simulink library "inp"  (R2021b)
settings: Solver=VariableStepAuto  StartTime=0.0  StopTime=10.0  RelTol=1e-3
undefined symbols (not defined in the file): C_TASK_5MS_S, FALSE, KINP_AcoreReadyToSlp_flg_ovrdflg, KINP_AcoreReadyToSlp_flg_ovrdval, KINP_AllowMovThd_OTA_enum_ovrdflg, KINP_AllowMovThd_OTA_enum_ovrdval, KINP_APSAngleTarget_Deg_ovrdflg, KINP_APSAngleTarget_Deg_ovrdval, KINP_APSDecReq_mps2_ovrdflg, KINP_APSDecReq_mps2_ovrdval, KINP_APSDecReqA_flg_ovrdflg, KINP_APSDecReqA_flg_ovrdval, KINP_APSDFLL_cm_ovrdflg, KINP_APSDFLL_cm_ovrdval, KINP_APSDFLR_cm_ovrdflg, KINP_APSDFLR_cm_ovrdval, KINP_APSDRLL_cm_ovrdflg, KINP_APSDRLL_cm_ovrdval, KINP_APSDRLR_cm_ovrdflg, KINP_APSDRLR_cm_ovrdval, KINP_APSExitCondition_enum_ovrdflg, KINP_APSExitCondition_enum_ovrdval, KINP_APSHWVer_enum_ovrdflg, KINP_APSHWVer_enum_ovrdval, KINP_APSProgressPCT_pct_ovrdflg, KINP_APSProgressPCT_pct_ovrdval, KINP_APSReq_enum_ovrdflg, KINP_APSReq_enum_ovrdval, KINP_APSRQDisplay_enum_ovrdflg, KINP_APSRQDisplay_enum_ovrdval, KINP_APSRqEPASCtrl_flg_ovrdflg, KINP_APSRqEPASCtrl_flg_ovrdval, KINP_APSShiftPosnReq_enum_ovrdval, KINP_APSShiftPosnReq_enum_ovrflg, KINP_APSSpeedCMD_kph_ovrdval, KINP_APSSpeedCMD_kph_ovrflg, KINP_APSStaSystem_enum_ovrdflg, KINP_APSStaSystem_enum_ovrdval, KINP_APSSWVer_enum_ovrdflg, KINP_APSSWVer_enum_ovrdval, KINP_APSVMCReqA_flg_ovrdval, KINP_APSVMCReqA_flg_ovrflg, KINP_APSVRqEPASCtrl_flg_ovrdflg, KINP_APSVRqEPASCtrl_flg_ovrdval, KINP_AuxBattVolmV_mV_ovrdflg, KINP_AuxBattVolmV_mV_ovrdval, KINP_CAASSta_enum_ovrdflg, KINP_CAASSta_enum_ovrdval, KINP_CAASVMCReqA_flg_ovrdval, KINP_CAASVMCReqA_flg_ovrflg, KINP_Chime_enum_ovrdflg, KINP_Chime_enum_ovrdval, KINP_ClearDTCcmd_flg_ovrdflg, KINP_ClearDTCcmd_flg_ovrdval, KINP_EvccAplusPwrUpReq_flg_ovrdflg, KINP_EvccAplusPwrUpReq_flg_ovrdval, KINP_LFID_raw_ovrdval, KINP_LFID_raw_ovrflg, KINP_LRID_raw_ovrdval, KINP_MemOffsetAccX_raw16_ovrdflg ... (+118)
libraries: FVT_lib x503, hcu_lib x1
(part 9 of 16)

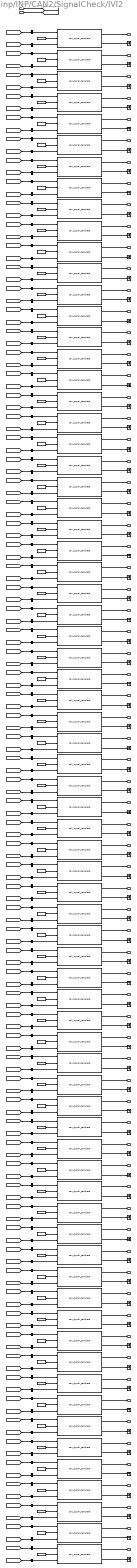
== system inp/INP/CAN2/SignalCheck/IVI2 ==
  BHAL_outputs : Inport
  inp_CanValid_bus : Inport  Port=2
  ACChgCurSet : FVT_lib/inp/can_signal_template  SystemSampleTime=-1  VariantActivationTime=update diagram  Latency=0  AutoFrameSizeCalculation=off
      link override defval: Value=KINP_ACChgCurSet_A_defval
      link override ovrdflg: Value=KINP_ACChgCurSet_A_ovrdflg
      link override ovrdval: Value=KINP_ACChgCurSet_A_ovrdval
  AVMErrSTA : FVT_lib/inp/can_signal_template  SystemSampleTime=-1  VariantActivationTime=update diagram  Latency=0  AutoFrameSizeCalculation=off
      link override defval: Value=KINP_AVMErrSTA_flg_defval
      link override ovrdflg: Value=KINP_AVMErrSTA_flg_ovrdflg
      link override ovrdval: Value=KINP_AVMErrSTA_flg_ovrdval
  AVMOFFRecButt : FVT_lib/inp/can_signal_template  SystemSampleTime=-1  VariantActivationTime=update diagram  Latency=0  AutoFrameSizeCalculation=off
      link override defval: Value=KINP_AVMOFFRecButt_flg_defval
      link override ovrdflg: Value=KINP_AVMOFFRecButt_flg_ovrdflg
      link override ovrdval: Value=KINP_AVMOFFRecButt_flg_ovrdval
  AVMParkingmode : FVT_lib/inp/can_signal_template  SystemSampleTime=-1  VariantActivationTime=update diagram  Latency=0  AutoFrameSizeCalculation=off
      link override defval: Value=KINP_AVMParkingmode_enum_defval
      link override ovrdflg: Value=KINP_AVMParkingmode_enum_ovrdflg
      link override ovrdval: Value=KINP_AVMParkingmode_enum_ovrdval
  AVMparkingcancel : FVT_lib/inp/can_signal_template  SystemSampleTime=-1  VariantActivationTime=update diagram  Latency=0  AutoFrameSizeCalculation=off
      link override defval: Value=KINP_AVMparkingcancel_enum_defval
      link override ovrdflg: Value=KINP_AVMparkingcancel_enum_ovrdflg
      link override ovrdval: Value=KINP_AVMparkingcancel_enum_ovrdval
  AVMparkingexcute : FVT_lib/inp/can_signal_template  SystemSampleTime=-1  VariantActivationTime=update diagram  Latency=0  AutoFrameSizeCalculation=off
      link override defval: Value=KINP_AVMparkingexcute_enum_defval
      link override ovrdflg: Value=KINP_AVMparkingexcute_enum_ovrdflg
      link override ovrdval: Value=KINP_AVMparkingexcute_enum_ovrdval
  CAASSw : FVT_lib/inp/can_signal_template  SystemSampleTime=-1  VariantActivationTime=update diagram  Latency=0  AutoFrameSizeCalculation=off
      link override defval: Value=KINP_CAASSw_enum_defval
      link override ovrdflg: Value=KINP_CAASSw_enum_ovrdflg
      link override ovrdval: Value=KINP_CAASSw_enum_ovrdval
  CDLLockButt : FVT_lib/inp/can_signal_template  SystemSampleTime=-1  VariantActivationTime=update diagram  Latency=0  AutoFrameSizeCalculation=off
      link override defval: Value=KINP_CDLLockButt_flg_defval
      link override ovrdflg: Value=KINP_CDLLockButt_flg_ovrdflg
      link override ovrdval: Value=KINP_CDLLockButt_flg_ovrdval
  CDLUnlockButt : FVT_lib/inp/can_signal_template  SystemSampleTime=-1  VariantActivationTime=update diagram  Latency=0  AutoFrameSizeCalculation=off
      link override defval: Value=KINP_CDLUnlockButt_flg_defval
      link override ovrdflg: Value=KINP_CDLUnlockButt_flg_ovrdflg
      link override ovrdval: Value=KINP_CDLUnlockButt_flg_ovrdval
  DSEATantiset : FVT_lib/inp/can_signal_template  SystemSampleTime=-1  VariantActivationTime=update diagram  Latency=0  AutoFrameSizeCalculation=off
      link override defval: Value=KINP_DSEATantiset_flg_defval
      link override ovrdflg: Value=KINP_DSEATantiset_flg_ovrdflg
      link override ovrdval: Value=KINP_DSEATantiset_flg_ovrdval
  DSEATentryfunset : FVT_lib/inp/can_signal_template  SystemSampleTime=-1  VariantActivationTime=update diagram  Latency=0  AutoFrameSizeCalculation=off
      link override defval: Value=KINP_DSEATentryfunset_flg_defval
      link override ovrdflg: Value=KINP_DSEATentryfunset_flg_ovrdflg
      link override ovrdval: Value=KINP_DSEATentryfunset_flg_ovrdval
  DSEATventreq : FVT_lib/inp/can_signal_template  SystemSampleTime=-1  VariantActivationTime=update diagram  Latency=0  AutoFrameSizeCalculation=off
      link override defval: Value=KINP_DSEATventreq_enum_defval
      link override ovrdflg: Value=KINP_DSEATventreq_enum_ovrdflg
      link override ovrdval: Value=KINP_DSEATventreq_enum_ovrdval
  Distanceunit : FVT_lib/inp/can_signal_template  SystemSampleTime=-1  VariantActivationTime=update diagram  Latency=0  AutoFrameSizeCalculation=off
      link override defval: Value=KINP_Distanceunit_flg_defval
      link override ovrdflg: Value=KINP_Distanceunit_flg_ovrdflg
      link override ovrdval: Value=KINP_Distanceunit_flg_ovrdval
  ESCSWCmd : FVT_lib/inp/can_signal_template  SystemSampleTime=-1  VariantActivationTime=update diagram  Latency=0  AutoFrameSizeCalculation=off
      link override defval: Value=KINP_ESCSWCmd_enum_defval
      link override ovrdflg: Value=KINP_ESCSWCmd_enum_ovrdflg
      link override ovrdval: Value=KINP_ESCSWCmd_enum_ovrdval
  FSOffSw : FVT_lib/inp/can_signal_template  SystemSampleTime=-1  VariantActivationTime=update diagram  Latency=0  AutoFrameSizeCalculation=off
      link override defval: Value=KINP_FSOffSw_enum_defval
      link override ovrdflg: Value=KINP_FSOffSw_enum_ovrdflg
      link override ovrdval: Value=KINP_FSOffSw_enum_ovrdval
  FollowMeSW : FVT_lib/inp/can_signal_template  SystemSampleTime=-1  VariantActivationTime=update diagram  Latency=0  AutoFrameSizeCalculation=off
      link override defval: Value=KINP_FollowMeSW_flg_defval
      link override ovrdflg: Value=KINP_FollowMeSW_flg_ovrdflg
      link override ovrdval: Value=KINP_FollowMeSW_flg_ovrdval
  GPSLAT : FVT_lib/inp/can_signal_template  SystemSampleTime=-1  VariantActivationTime=update diagram  Latency=0  AutoFrameSizeCalculation=off
      link override defval: Value=KINP_GPSLAT_s_defval
      link override ovrdflg: Value=KINP_GPSLAT_s_ovrdflg
      link override ovrdval: Value=KINP_GPSLAT_s_ovrdval
  GPSLONG : FVT_lib/inp/can_signal_template  SystemSampleTime=-1  VariantActivationTime=update diagram  Latency=0  AutoFrameSizeCalculation=off
      link override defval: Value=KINP_GPSLONG_enum_defval
      link override ovrdflg: Value=KINP_GPSLONG_enum_ovrdflg
      link override ovrdval: Value=KINP_GPSLONG_enum_ovrdval
  HeadLampSW : FVT_lib/inp/can_signal_template  SystemSampleTime=-1  VariantActivationTime=update diagram  Latency=0  AutoFrameSizeCalculation=off
      link override defval: Value=KINP_HeadLampSW_enum_defval
      link override ovrdflg: Value=KINP_HeadLampSW_enum_ovrdflg
      link override ovrdval: Value=KINP_HeadLampSW_enum_ovrdval
  HoodLatchSW : FVT_lib/inp/can_signal_template  SystemSampleTime=-1  VariantActivationTime=update diagram  Latency=0  AutoFrameSizeCalculation=off
      link override defval: Value=KINP_HoodLatchSW_enum_defval
      link override ovrdflg: Value=KINP_HoodLatchSW_enum_ovrdflg
      link override ovrdval: Value=KINP_HoodLatchSW_enum_ovrdval
  IVINightModeSta : FVT_lib/inp/can_signal_template  SystemSampleTime=-1  VariantActivationTime=update diagram  Latency=0  AutoFrameSizeCalculation=off
      link override defval: Value=KINP_IVINightModeSta_flg_defval
      link override ovrdflg: Value=KINP_IVINightModeSta_flg_ovrdflg
      link override ovrdval: Value=KINP_IVINightModeSta_flg_ovrdval
  IVIPTGModeSW : FVT_lib/inp/can_signal_template  SystemSampleTime=-1  VariantActivationTime=update diagram  Latency=0  AutoFrameSizeCalculation=off
      link override defval: Value=KINP_IVIPTGModeSW_enum_defval
      link override ovrdflg: Value=KINP_IVIPTGModeSW_enum_ovrdflg
      link override ovrdval: Value=KINP_IVIPTGModeSW_enum_ovrdval
  IVIPTGStaSW : FVT_lib/inp/can_signal_template  SystemSampleTime=-1  VariantActivationTime=update diagram  Latency=0  AutoFrameSizeCalculation=off
      link override defval: Value=KINP_IVIPTGStaSW_enum_defval
      link override ovrdflg: Value=KINP_IVIPTGStaSW_enum_ovrdflg
      link override ovrdval: Value=KINP_IVIPTGStaSW_enum_ovrdval
  IVIPTGUSStaSW : FVT_lib/inp/can_signal_template  SystemSampleTime=-1  VariantActivationTime=update diagram  Latency=0  AutoFrameSizeCalculation=off
      link override defval: Value=KINP_IVIPTGUSStaSW_flg_defval
      link override ovrdflg: Value=KINP_IVIPTGUSStaSW_flg_ovrdflg
      link override ovrdval: Value=KINP_IVIPTGUSStaSW_flg_ovrdval
  IVIPWModeReq : FVT_lib/inp/can_signal_template  SystemSampleTime=-1  VariantActivationTime=update diagram  Latency=0  AutoFrameSizeCalculation=off
      link override defval: Value=KINP_IVIPWModeReq_enum_defval
      link override ovrdflg: Value=KINP_IVIPWModeReq_enum_ovrdflg
      link override ovrdval: Value=KINP_IVIPWModeReq_enum_ovrdval
  IVIPwrLockSW : FVT_lib/inp/can_signal_template  SystemSampleTime=-1  VariantActivationTime=update diagram  Latency=0  AutoFrameSizeCalculation=off
      link override defval: Value=KINP_IVIPwrLockSW_enum_defval
      link override ovrdflg: Value=KINP_IVIPwrLockSW_enum_ovrdflg
      link override ovrdval: Value=KINP_IVIPwrLockSW_enum_ovrdval
  IVIPwroffreq : FVT_lib/inp/can_signal_template  SystemSampleTime=-1  VariantActivationTime=update diagram  Latency=0  AutoFrameSizeCalculation=off
      link override defval: Value=KINP_IVIPwroffreq_flg_defval
      link override ovrdflg: Value=KINP_IVIPwroffreq_flg_ovrdflg
      link override ovrdval: Value=KINP_IVIPwroffreq_flg_ovrdval
  IVIRRDefReq : FVT_lib/inp/can_signal_template  SystemSampleTime=-1  VariantActivationTime=update diagram  Latency=0  AutoFrameSizeCalculation=off
      link override defval: Value=KINP_IVIRRDefReq_flg_defval
      link override ovrdflg: Value=KINP_IVIRRDefReq_flg_ovrdflg
      link override ovrdval: Value=KINP_IVIRRDefReq_flg_ovrdval
  IVIReqV2L : FVT_lib/inp/can_signal_template  SystemSampleTime=-1  VariantActivationTime=update diagram  Latency=0  AutoFrameSizeCalculation=off
      link override defval: Value=KINP_IVIReqV2L_enum_defval
      link override ovrdflg: Value=KINP_IVIReqV2L_enum_ovrdflg
      link override ovrdval: Value=KINP_IVIReqV2L_enum_ovrdval
  IVIScreen : FVT_lib/inp/can_signal_template  SystemSampleTime=-1  VariantActivationTime=update diagram  Latency=0  AutoFrameSizeCalculation=off
      link override defval: Value=KINP_IVIScreen_enum_defval
      link override ovrdflg: Value=KINP_IVIScreen_enum_ovrdflg
      link override ovrdval: Value=KINP_IVIScreen_enum_ovrdval
  IVIStartChgreq : FVT_lib/inp/can_signal_template  SystemSampleTime=-1  VariantActivationTime=update diagram  Latency=0  AutoFrameSizeCalculation=off
      link override defval: Value=KINP_IVIStartChgreq_flg_defval
      link override ovrdflg: Value=KINP_IVIStartChgreq_flg_ovrdflg
      link override ovrdval: Value=KINP_IVIStartChgreq_flg_ovrdval
  IVIStatus : FVT_lib/inp/can_signal_template  SystemSampleTime=-1  VariantActivationTime=update diagram  Latency=0  AutoFrameSizeCalculation=off
      link override defval: Value=KINP_IVIStatus_flg_defval
      link override ovrdflg: Value=KINP_IVIStatus_flg_ovrdflg
      link override ovrdval: Value=KINP_IVIStatus_flg_ovrdval
  IVIStopChgreq : FVT_lib/inp/can_signal_template  SystemSampleTime=-1  VariantActivationTime=update diagram  Latency=0  AutoFrameSizeCalculation=off
      link override defval: Value=KINP_IVIStopChgreq_flg_defval
      link override ovrdflg: Value=KINP_IVIStopChgreq_flg_ovrdflg
      link override ovrdval: Value=KINP_IVIStopChgreq_flg_ovrdval
  IVITriggerreq : FVT_lib/inp/can_signal_template  SystemSampleTime=-1  VariantActivationTime=update diagram  Latency=0  AutoFrameSizeCalculation=off
      link override defval: Value=KINP_IVITriggerreq_flg_defval
      link override ovrdflg: Value=KINP_IVITriggerreq_flg_ovrdflg
      link override ovrdval: Value=KINP_IVITriggerreq_flg_ovrdval
  IVIUnlockChgreq : FVT_lib/inp/can_signal_template  SystemSampleTime=-1  VariantActivationTime=update diagram  Latency=0  AutoFrameSizeCalculation=off
      link override defval: Value=KINP_IVIUnlockChgreq_flg_defval
      link override ovrdflg: Value=KINP_IVIUnlockChgreq_flg_ovrdflg
      link override ovrdval: Value=KINP_IVIUnlockChgreq_flg_ovrdval
  IVIWIMAINSW : FVT_lib/inp/can_signal_template  SystemSampleTime=-1  VariantActivationTime=update diagram  Latency=0  AutoFrameSizeCalculation=off
      link override defval: Value=KINP_IVIWIMAINSW_flg_defval
      link override ovrdflg: Value=KINP_IVIWIMAINSW_flg_ovrdflg
      link override ovrdval: Value=KINP_IVIWIMAINSW_flg_ovrdval
  LDrvControlCommand : FVT_lib/inp/can_signal_template  SystemSampleTime=-1  VariantActivationTime=update diagram  Latency=0  AutoFrameSizeCalculation=off
      link override defval: Value=KINP_LDrvControlCommand_pct_defval
      link override ovrdflg: Value=KINP_LDrvControlCommand_pct_ovrdflg
      link override ovrdval: Value=KINP_LDrvControlCommand_pct_ovrdval
  LPasControlCommand : FVT_lib/inp/can_signal_template  SystemSampleTime=-1  VariantActivationTime=update diagram  Latency=0  AutoFrameSizeCalculation=off
      link override defval: Value=KINP_LPasControlCommand_pct_defval
      link override ovrdflg: Value=KINP_LPasControlCommand_pct_ovrdflg
      link override ovrdval: Value=KINP_LPasControlCommand_pct_ovrdval
  LRLDControlCommand : FVT_lib/inp/can_signal_template  SystemSampleTime=-1  VariantActivationTime=update diagram  Latency=0  AutoFrameSizeCalculation=off
      link override defval: Value=KINP_LRLDControlCommand_pct_defval
      link override ovrdflg: Value=KINP_LRLDControlCommand_pct_ovrdflg
      link override ovrdval: Value=KINP_LRLDControlCommand_pct_ovrdval
  LRRDControlCommand : FVT_lib/inp/can_signal_template  SystemSampleTime=-1  VariantActivationTime=update diagram  Latency=0  AutoFrameSizeCalculation=off
      link override defval: Value=KINP_LRRDControlCommand_pct_defval
      link override ovrdflg: Value=KINP_LRRDControlCommand_pct_ovrdflg
      link override ovrdval: Value=KINP_LRRDControlCommand_pct_ovrdval
  LightShowStartReq : FVT_lib/inp/can_signal_template  SystemSampleTime=-1  VariantActivationTime=update diagram  Latency=0  AutoFrameSizeCalculation=off
      link override defval: Value=KINP_LightShowStartReq_flg_defval
      link override ovrdflg: Value=KINP_LightShowStartReq_flg_ovrdflg
      link override ovrdval: Value=KINP_LightShowStartReq_flg_ovrdval
  LightShowStopReq : FVT_lib/inp/can_signal_template  SystemSampleTime=-1  VariantActivationTime=update diagram  Latency=0  AutoFrameSizeCalculation=off
      link override defval: Value=KINP_LightShowStopReq_flg_defval
      link override ovrdflg: Value=KINP_LightShowStopReq_flg_ovrdflg
      link override ovrdval: Value=KINP_LightShowStopReq_flg_ovrdval
  MFRDNBrightReq : FVT_lib/inp/can_signal_template  SystemSampleTime=-1  VariantActivationTime=update diagram  Latency=0  AutoFrameSizeCalculation=off
      link override defval: Value=KINP_MFRDNBrightReq_pct_defval
      link override ovrdflg: Value=KINP_MFRDNBrightReq_pct_ovrdflg
      link override ovrdval: Value=KINP_MFRDNBrightReq_pct_ovrdval
  OFFACMODE : FVT_lib/inp/can_signal_template  SystemSampleTime=-1  VariantActivationTime=update diagram  Latency=0  AutoFrameSizeCalculation=off
      link override defval: Value=KINP_OFFACMODE_enum_defval
      link override ovrdflg: Value=KINP_OFFACMODE_enum_ovrdflg
      link override ovrdval: Value=KINP_OFFACMODE_enum_ovrdval
  PSEATventreq : FVT_lib/inp/can_signal_template  SystemSampleTime=-1  VariantActivationTime=update diagram  Latency=0  AutoFrameSizeCalculation=off
      link override defval: Value=KINP_PSEATventreq_enum_defval
      link override ovrdflg: Value=KINP_PSEATventreq_enum_ovrdflg
      link override ovrdval: Value=KINP_PSEATventreq_enum_ovrdval
  PerdV2L : FVT_lib/inp/can_signal_template  SystemSampleTime=-1  VariantActivationTime=update diagram  Latency=0  AutoFrameSizeCalculation=off
      link override defval: Value=KINP_PerdV2L_enum_defval
      link override ovrdflg: Value=KINP_PerdV2L_enum_ovrdflg
      link override ovrdval: Value=KINP_PerdV2L_enum_ovrdval
  RFogLampSW : FVT_lib/inp/can_signal_template  SystemSampleTime=-1  VariantActivationTime=update diagram  Latency=0  AutoFrameSizeCalculation=off
      link override defval: Value=KINP_RFogLampSW_flg_defval
      link override ovrdflg: Value=KINP_RFogLampSW_flg_ovrdflg
      link override ovrdval: Value=KINP_RFogLampSW_flg_ovrdval
  RollModeSWCmd : FVT_lib/inp/can_signal_template  SystemSampleTime=-1  VariantActivationTime=update diagram  Latency=0  AutoFrameSizeCalculation=off
      link override defval: Value=KINP_RollModeSWCmd_enum_defval
      link override ovrdflg: Value=KINP_RollModeSWCmd_enum_ovrdflg
      link override ovrdval: Value=KINP_RollModeSWCmd_enum_ovrdval
  RoomLampMode : FVT_lib/inp/can_signal_template  SystemSampleTime=-1  VariantActivationTime=update diagram  Latency=0  AutoFrameSizeCalculation=off
      link override defval: Value=KINP_RoomLampMode_flg_defval
      link override ovrdflg: Value=KINP_RoomLampMode_flg_ovrdflg
      link override ovrdval: Value=KINP_RoomLampMode_flg_ovrdval
  SOCADJBUTT : FVT_lib/inp/can_signal_template  SystemSampleTime=-1  VariantActivationTime=update diagram  Latency=0  AutoFrameSizeCalculation=off
      link override defval: Value=KINP_SOCADJBUTT_flg_defval
      link override ovrdflg: Value=KINP_SOCADJBUTT_flg_ovrdflg
      link override ovrdval: Value=KINP_SOCADJBUTT_flg_ovrdval
  SOCLimitSet : FVT_lib/inp/can_signal_template  SystemSampleTime=-1  VariantActivationTime=update diagram  Latency=0  AutoFrameSizeCalculation=off
      link override defval: Value=KINP_SOCLimitSet_pct_defval
      link override ovrdflg: Value=KINP_SOCLimitSet_pct_ovrdflg
      link override ovrdval: Value=KINP_SOCLimitSet_pct_ovrdval
  SOCV2LLimit : FVT_lib/inp/can_signal_template  SystemSampleTime=-1  VariantActivationTime=update diagram  Latency=0  AutoFrameSizeCalculation=off
      link override defval: Value=KINP_SOCV2LLimit_pct_defval
      link override ovrdflg: Value=KINP_SOCV2LLimit_pct_ovrdflg
      link override ovrdval: Value=KINP_SOCV2LLimit_pct_ovrdval
  SchedChgStart : FVT_lib/inp/can_signal_template  SystemSampleTime=-1  VariantActivationTime=update diagram  Latency=0  AutoFrameSizeCalculation=off
      link override defval: Value=KINP_SchedChgStart_flg_defval
      link override ovrdflg: Value=KINP_SchedChgStart_flg_ovrdflg
      link override ovrdval: Value=KINP_SchedChgStart_flg_ovrdval
  SchedChgStop : FVT_lib/inp/can_signal_template  SystemSampleTime=-1  VariantActivationTime=update diagram  Latency=0  AutoFrameSizeCalculation=off
      link override defval: Value=KINP_SchedChgStop_flg_defval
      link override ovrdflg: Value=KINP_SchedChgStop_flg_ovrdflg
      link override ovrdval: Value=KINP_SchedChgStop_flg_ovrdval
  SchedChgbutt : FVT_lib/inp/can_signal_template  SystemSampleTime=-1  VariantActivationTime=update diagram  Latency=0  AutoFrameSizeCalculation=off
      link override defval: Value=KINP_SchedChgbutt_flg_defval
      link override ovrdflg: Value=KINP_SchedChgbutt_flg_ovrdflg
      link override ovrdval: Value=KINP_SchedChgbutt_flg_ovrdval
  SchedChglimit : FVT_lib/inp/can_signal_template  SystemSampleTime=-1  VariantActivationTime=update diagram  Latency=0  AutoFrameSizeCalculation=off
      link override defval: Value=KINP_SchedChglimit_pct_defval
      link override ovrdflg: Value=KINP_SchedChglimit_pct_ovrdflg
      link override ovrdval: Value=KINP_SchedChglimit_pct_ovrdval
  SchedChgwake : FVT_lib/inp/can_signal_template  SystemSampleTime=-1  VariantActivationTime=update diagram  Latency=0  AutoFrameSizeCalculation=off
      link override defval: Value=KINP_SchedChgwake_flg_defval
      link override ovrdflg: Value=KINP_SchedChgwake_flg_ovrdflg
      link override ovrdval: Value=KINP_SchedChgwake_flg_ovrdval
  SenstivityPosition : FVT_lib/inp/can_signal_template  SystemSampleTime=-1  VariantActivationTime=update diagram  Latency=0  AutoFrameSizeCalculation=off
      link override defval: Value=KINP_SenstivityPosition_enum_defval
      link override ovrdflg: Value=KINP_SenstivityPosition_enum_ovrdflg
      link override ovrdval: Value=KINP_SenstivityPosition_enum_ovrdval
  SetUnlockSingle : FVT_lib/inp/can_signal_template  SystemSampleTime=-1  VariantActivationTime=update diagram  Latency=0  AutoFrameSizeCalculation=off
      link override defval: Value=KINP_SetUnlockSingle_flg_defval
      link override ovrdflg: Value=KINP_SetUnlockSingle_flg_ovrdflg
      link override ovrdval: Value=KINP_SetUnlockSingle_flg_ovrdval
  TCSSWCmd : FVT_lib/inp/can_signal_template  SystemSampleTime=-1  VariantActivationTime=update diagram  Latency=0  AutoFrameSizeCalculation=off
      link override defval: Value=KINP_TCSSWCmd_enum_defval
      link override ovrdflg: Value=KINP_TCSSWCmd_enum_ovrdflg
      link override ovrdval: Value=KINP_TCSSWCmd_enum_ovrdval
  TPMSCaliButt : FVT_lib/inp/can_signal_template  SystemSampleTime=-1  VariantActivationTime=update diagram  Latency=0  AutoFrameSizeCalculation=off
      link override defval: Value=KINP_TPMSCaliButt_flg_defval
      link override ovrdflg: Value=KINP_TPMSCaliButt_flg_ovrdflg
      link override ovrdval: Value=KINP_TPMSCaliButt_flg_ovrdval
  TPMSResButt : FVT_lib/inp/can_signal_template  SystemSampleTime=-1  VariantActivationTime=update diagram  Latency=0  AutoFrameSizeCalculation=off
      link override defval: Value=KINP_TPMSResButt_flg_defval
      link override ovrdflg: Value=KINP_TPMSResButt_flg_ovrdflg
      link override ovrdval: Value=KINP_TPMSResButt_flg_ovrdval
  Terminator_{1..72} (72 alike) : Terminator
  True_VHAL_ACChgCurSet_A : Constant  Value=TRUE  OutDataTypeStr=boolean
  True_VHAL_AVMErrSTA_flg : Constant  Value=TRUE  OutDataTypeStr=boolean
  True_VHAL_AVMOFFRecButt_flg : Constant  Value=TRUE  OutDataTypeStr=boolean
  True_VHAL_AVMParkingmode_enum : Constant  Value=TRUE  OutDataTypeStr=boolean
  True_VHAL_AVMparkingcancel_enum : Constant  Value=TRUE  OutDataTypeStr=boolean
  True_VHAL_AVMparkingexcute_enum : Constant  Value=TRUE  OutDataTypeStr=boolean
  True_VHAL_CAASSw_enum : Constant  Value=TRUE  OutDataTypeStr=boolean
  True_VHAL_CDLLockButt_flg : Constant  Value=TRUE  OutDataTypeStr=boolean
  True_VHAL_CDLUnlockButt_flg : Constant  Value=TRUE  OutDataTypeStr=boolean
  True_VHAL_DSEATantiset_flg : Constant  Value=TRUE  OutDataTypeStr=boolean
  True_VHAL_DSEATentryfunset_flg : Constant  Value=TRUE  OutDataTypeStr=boolean
  True_VHAL_DSEATventreq_enum : Constant  Value=TRUE  OutDataTypeStr=boolean
  True_VHAL_Distanceunit_flg : Constant  Value=TRUE  OutDataTypeStr=boolean
  True_VHAL_ESCSWCmd_enum : Constant  Value=TRUE  OutDataTypeStr=boolean
  True_VHAL_FSOffSw_enum : Constant  Value=TRUE  OutDataTypeStr=boolean
  True_VHAL_FollowMeSW_flg : Constant  Value=TRUE  OutDataTypeStr=boolean
  True_VHAL_GPSLAT_s : Constant  Value=TRUE  OutDataTypeStr=boolean
  True_VHAL_GPSLONG_enum : Constant  Value=TRUE  OutDataTypeStr=boolean
  True_VHAL_HeadLampSW_enum : Constant  Value=TRUE  OutDataTypeStr=boolean
  True_VHAL_HoodLatchSW_enum : Constant  Value=TRUE  OutDataTypeStr=boolean
  True_VHAL_IVINightModeSta_flg : Constant  Value=TRUE  OutDataTypeStr=boolean
  True_VHAL_IVIPTGModeSW_enum : Constant  Value=TRUE  OutDataTypeStr=boolean
  True_VHAL_IVIPTGStaSW_enum : Constant  Value=TRUE  OutDataTypeStr=boolean
  True_VHAL_IVIPTGUSStaSW_flg : Constant  Value=TRUE  OutDataTypeStr=boolean
  True_VHAL_IVIPWModeReq_enum : Constant  Value=TRUE  OutDataTypeStr=boolean
  True_VHAL_IVIPwrLockSW_enum : Constant  Value=TRUE  OutDataTypeStr=boolean
  True_VHAL_IVIPwroffreq_flg : Constant  Value=TRUE  OutDataTypeStr=boolean
  True_VHAL_IVIRRDefReq_flg : Constant  Value=TRUE  OutDataTypeStr=boolean
  True_VHAL_IVIReqV2L_enum : Constant  Value=TRUE  OutDataTypeStr=boolean
  True_VHAL_IVIScreen_enum : Constant  Value=TRUE  OutDataTypeStr=boolean
  True_VHAL_IVIStartChgreq_flg : Constant  Value=TRUE  OutDataTypeStr=boolean
  True_VHAL_IVIStatus_flg : Constant  Value=TRUE  OutDataTypeStr=boolean
  True_VHAL_IVIStopChgreq_flg : Constant  Value=TRUE  OutDataTypeStr=boolean
  True_VHAL_IVITriggerreq_flg : Constant  Value=TRUE  OutDataTypeStr=boolean
  True_VHAL_IVIUnlockChgreq_flg : Constant  Value=TRUE  OutDataTypeStr=boolean
  True_VHAL_IVIWIMAINSW_flg : Constant  Value=TRUE  OutDataTypeStr=boolean
  True_VHAL_LDrvControlCommand_pct : Constant  Value=TRUE  OutDataTypeStr=boolean
  True_VHAL_LPasControlCommand_pct : Constant  Value=TRUE  OutDataTypeStr=boolean
  True_VHAL_LRLDControlCommand_pct : Constant  Value=TRUE  OutDataTypeStr=boolean
  True_VHAL_LRRDControlCommand_pct : Constant  Value=TRUE  OutDataTypeStr=boolean
  True_VHAL_LightShowStartReq_flg : Constant  Value=TRUE  OutDataTypeStr=boolean
  True_VHAL_LightShowStopReq_flg : Constant  Value=TRUE  OutDataTypeStr=boolean
  True_VHAL_MFRDNBrightReq_pct : Constant  Value=TRUE  OutDataTypeStr=boolean
  True_VHAL_OFFACMODE_enum : Constant  Value=TRUE  OutDataTypeStr=boolean
  True_VHAL_PSEATventreq_enum : Constant  Value=TRUE  OutDataTypeStr=boolean
  True_VHAL_PerdV2L_enum : Constant  Value=TRUE  OutDataTypeStr=boolean
  True_VHAL_RFogLampSW_flg : Constant  Value=TRUE  OutDataTypeStr=boolean
  True_VHAL_RollModeSWCmd_enum : Constant  Value=TRUE  OutDataTypeStr=boolean
  True_VHAL_RoomLampMode_flg : Constant  Value=TRUE  OutDataTypeStr=boolean
  True_VHAL_SOCADJBUTT_flg : Constant  Value=TRUE  OutDataTypeStr=boolean
  True_VHAL_SOCLimitSet_pct : Constant  Value=TRUE  OutDataTypeStr=boolean
  True_VHAL_SOCV2LLimit_pct : Constant  Value=TRUE  OutDataTypeStr=boolean
  True_VHAL_SchedChgStart_flg : Constant  Value=TRUE  OutDataTypeStr=boolean
  True_VHAL_SchedChgStop_flg : Constant  Value=TRUE  OutDataTypeStr=boolean
  True_VHAL_SchedChgbutt_flg : Constant  Value=TRUE  OutDataTypeStr=boolean
  True_VHAL_SchedChglimit_pct : Constant  Value=TRUE  OutDataTypeStr=boolean
  True_VHAL_SchedChgwake_flg : Constant  Value=TRUE  OutDataTypeStr=boolean
  True_VHAL_SenstivityPosition_enum : Constant  Value=TRUE  OutDataTypeStr=boolean
  True_VHAL_SetUnlockSingle_flg : Constant  Value=TRUE  OutDataTypeStr=boolean
  True_VHAL_TCSSWCmd_enum : Constant  Value=TRUE  OutDataTypeStr=boolean
  True_VHAL_TPMSCaliButt_flg : Constant  Value=TRUE  OutDataTypeStr=boolean
  True_VHAL_TPMSResButt_flg : Constant  Value=TRUE  OutDataTypeStr=boolean
  True_VHAL_TurnSwTimeSet_enum : Constant  Value=TRUE  OutDataTypeStr=boolean
  True_VHAL_WalkawayLockSW_flg : Constant  Value=TRUE  OutDataTypeStr=boolean
  True_VHAL_WlcmLightMode_enum : Constant  Value=TRUE  OutDataTypeStr=boolean
  True_VHAL_sigAirIntenZon1Req_enum : Constant  Value=TRUE  OutDataTypeStr=boolean
  True_VHAL_sigDfrstReq_flg : Constant  Value=TRUE  OutDataTypeStr=boolean
  True_VHAL_sigFaceReq_flg : Constant  Value=TRUE  OutDataTypeStr=boolean
  True_VHAL_sigFootReq_flg : Constant  Value=TRUE  OutDataTypeStr=boolean
  True_VHAL_sigRecircReq_flg : Constant  Value=TRUE  OutDataTypeStr=boolean
  True_VHAL_sigSetTempZon1Req_C : Constant  Value=TRUE  OutDataTypeStr=boolean
  True_VHAL_sigSetTempZon2Req_C : Constant  Value=TRUE  OutDataTypeStr=boolean
  TurnSwTimeSet : FVT_lib/inp/can_signal_template  SystemSampleTime=-1  VariantActivationTime=update diagram  Latency=0  AutoFrameSizeCalculation=off
      link override defval: Value=KINP_TurnSwTimeSet_enum_defval
      link override ovrdflg: Value=KINP_TurnSwTimeSet_enum_ovrdflg
      link override ovrdval: Value=KINP_TurnSwTimeSet_enum_ovrdval
  WalkawayLockSW : FVT_lib/inp/can_signal_template  SystemSampleTime=-1  VariantActivationTime=update diagram  Latency=0  AutoFrameSizeCalculation=off
      link override defval: Value=KINP_WalkawayLockSW_flg_defval
      link override ovrdflg: Value=KINP_WalkawayLockSW_flg_ovrdflg
      link override ovrdval: Value=KINP_WalkawayLockSW_flg_ovrdval
  WlcmLightMode : FVT_lib/inp/can_signal_template  SystemSampleTime=-1  VariantActivationTime=update diagram  Latency=0  AutoFrameSizeCalculation=off
      link override defval: Value=KINP_WlcmLightMode_enum_defval
      link override ovrdflg: Value=KINP_WlcmLightMode_enum_ovrdflg
      link override ovrdval: Value=KINP_WlcmLightMode_enum_ovrdval
  sigAirIntenZon1Req : FVT_lib/inp/can_signal_template  SystemSampleTime=-1  VariantActivationTime=update diagram  Latency=0  AutoFrameSizeCalculation=off
      link override defval: Value=KINP_sigAirIntenZon1Req_enum_defval
      link override ovrdflg: Value=KINP_sigAirIntenZon1Req_enum_ovrdflg
      link override ovrdval: Value=KINP_sigAirIntenZon1Req_enum_ovrdval
  sigDfrstReq : FVT_lib/inp/can_signal_template  SystemSampleTime=-1  VariantActivationTime=update diagram  Latency=0  AutoFrameSizeCalculation=off
      link override defval: Value=KINP_sigDfrstReq_flg_defval
      link override ovrdflg: Value=KINP_sigDfrstReq_flg_ovrdflg
      link override ovrdval: Value=KINP_sigDfrstReq_flg_ovrdval
  sigFaceReq : FVT_lib/inp/can_signal_template  SystemSampleTime=-1  VariantActivationTime=update diagram  Latency=0  AutoFrameSizeCalculation=off
      link override defval: Value=KINP_sigFaceReq_flg_defval
      link override ovrdflg: Value=KINP_sigFaceReq_flg_ovrdflg
      link override ovrdval: Value=KINP_sigFaceReq_flg_ovrdval
  sigFootReq : FVT_lib/inp/can_signal_template  SystemSampleTime=-1  VariantActivationTime=update diagram  Latency=0  AutoFrameSizeCalculation=off
      link override defval: Value=KINP_sigFootReq_flg_defval
      link override ovrdflg: Value=KINP_sigFootReq_flg_ovrdflg
      link override ovrdval: Value=KINP_sigFootReq_flg_ovrdval
  sigRecircReq : FVT_lib/inp/can_signal_template  SystemSampleTime=-1  VariantActivationTime=update diagram  Latency=0  AutoFrameSizeCalculation=off
      link override defval: Value=KINP_sigRecircReq_flg_defval
      link override ovrdflg: Value=KINP_sigRecircReq_flg_ovrdflg
      link override ovrdval: Value=KINP_sigRecircReq_flg_ovrdval
  sigSetTempZon1Req : FVT_lib/inp/can_signal_template  SystemSampleTime=-1  VariantActivationTime=update diagram  Latency=0  AutoFrameSizeCalculation=off
      link override defval: Value=KINP_sigSetTempZon1Req_C_defval
      link override ovrdflg: Value=KINP_sigSetTempZon1Req_C_ovrdflg
      link override ovrdval: Value=KINP_sigSetTempZon1Req_C_ovrdval
  sigSetTempZon2Req : FVT_lib/inp/can_signal_template  SystemSampleTime=-1  VariantActivationTime=update diagram  Latency=0  AutoFrameSizeCalculation=off
      link override defval: Value=KINP_sigSetTempZon2Req_C_defval
      link override ovrdflg: Value=KINP_sigSetTempZon2Req_C_ovrdflg
      link override ovrdval: Value=KINP_sigSetTempZon2Req_C_ovrdval
  slr1_{1..72} (72 alike) : BusSelector  OutputSignals=VINP_CANMsgValidIVI2_flg
  slr_VHAL_ACChgCurSet_A : BusSelector  OutputSignals=VHAL_ACChgCurSet_A
  slr_VHAL_AVMErrSTA_flg : BusSelector  OutputSignals=VHAL_AVMErrSTA_flg
  slr_VHAL_AVMOFFRecButt_flg : BusSelector  OutputSignals=VHAL_AVMOFFRecButt_flg
  slr_VHAL_AVMParkingmode_enum : BusSelector  OutputSignals=VHAL_AVMParkingmode_enum
  slr_VHAL_AVMparkingcancel_enum : BusSelector  OutputSignals=VHAL_AVMparkingcancel_enum
  slr_VHAL_AVMparkingexcute_enum : BusSelector  OutputSignals=VHAL_AVMparkingexcute_enum
  slr_VHAL_CAASSw_enum : BusSelector  OutputSignals=VHAL_CAASSw_enum
  slr_VHAL_CDLLockButt_flg : BusSelector  OutputSignals=VHAL_CDLLockButt_flg
  slr_VHAL_CDLUnlockButt_flg : BusSelector  OutputSignals=VHAL_CDLUnlockButt_flg
  slr_VHAL_DSEATantiset_flg : BusSelector  OutputSignals=VHAL_DSEATantiset_flg
  slr_VHAL_DSEATentryfunset_flg : BusSelector  OutputSignals=VHAL_DSEATentryfunset_flg
  slr_VHAL_DSEATventreq_enum : BusSelector  OutputSignals=VHAL_DSEATventreq_enum
  slr_VHAL_Distanceunit_flg : BusSelector  OutputSignals=VHAL_Distanceunit_flg
  slr_VHAL_ESCSWCmd_enum : BusSelector  OutputSignals=VHAL_ESCSWCmd_enum
  slr_VHAL_FSOffSw_enum : BusSelector  OutputSignals=VHAL_FSOffSw_enum
  slr_VHAL_FollowMeSW_flg : BusSelector  OutputSignals=VHAL_FollowMeSW_flg
  slr_VHAL_GPSLAT_s : BusSelector  OutputSignals=VHAL_GPSLAT_s
  slr_VHAL_GPSLONG_enum : BusSelector  OutputSignals=VHAL_GPSLONG_enum
  slr_VHAL_HeadLampSW_enum : BusSelector  OutputSignals=VHAL_HeadLampSW_enum
  slr_VHAL_HoodLatchSW_enum : BusSelector  OutputSignals=VHAL_HoodLatchSW_enum
  slr_VHAL_IVINightModeSta_flg : BusSelector  OutputSignals=VHAL_IVINightModeSta_flg
  slr_VHAL_IVIPTGModeSW_enum : BusSelector  OutputSignals=VHAL_IVIPTGModeSW_enum
  slr_VHAL_IVIPTGStaSW_enum : BusSelector  OutputSignals=VHAL_IVIPTGStaSW_enum
  slr_VHAL_IVIPTGUSStaSW_flg : BusSelector  OutputSignals=VHAL_IVIPTGUSStaSW_flg
  slr_VHAL_IVIPWModeReq_enum : BusSelector  OutputSignals=VHAL_IVIPWModeReq_enum
  slr_VHAL_IVIPwrLockSW_enum : BusSelector  OutputSignals=VHAL_IVIPwrLockSW_enum
  slr_VHAL_IVIPwroffreq_flg : BusSelector  OutputSignals=VHAL_IVIPwroffreq_flg
  slr_VHAL_IVIRRDefReq_flg : BusSelector  OutputSignals=VHAL_IVIRRDefReq_flg
  slr_VHAL_IVIReqV2L_enum : BusSelector  OutputSignals=VHAL_IVIReqV2L_enum
  slr_VHAL_IVIScreen_enum : BusSelector  OutputSignals=VHAL_IVIScreen_enum
  slr_VHAL_IVIStartChgreq_flg : BusSelector  OutputSignals=VHAL_IVIStartChgreq_flg
  slr_VHAL_IVIStatus_flg : BusSelector  OutputSignals=VHAL_IVIStatus_flg
  slr_VHAL_IVIStopChgreq_flg : BusSelector  OutputSignals=VHAL_IVIStopChgreq_flg
  slr_VHAL_IVITriggerreq_flg : BusSelector  OutputSignals=VHAL_IVITriggerreq_flg
  slr_VHAL_IVIUnlockChgreq_flg : BusSelector  OutputSignals=VHAL_IVIUnlockChgreq_flg
  slr_VHAL_IVIWIMAINSW_flg : BusSelector  OutputSignals=VHAL_IVIWIMAINSW_flg
  slr_VHAL_LDrvControlCommand_pct : BusSelector  OutputSignals=VHAL_LDrvControlCommand_pct
  slr_VHAL_LPasControlCommand_pct : BusSelector  OutputSignals=VHAL_LPasControlCommand_pct
  slr_VHAL_LRLDControlCommand_pct : BusSelector  OutputSignals=VHAL_LRLDControlCommand_pct
  slr_VHAL_LRRDControlCommand_pct : BusSelector  OutputSignals=VHAL_LRRDControlCommand_pct
  slr_VHAL_LightShowStartReq_flg : BusSelector  OutputSignals=VHAL_LightShowStartReq_flg
  slr_VHAL_LightShowStopReq_flg : BusSelector  OutputSignals=VHAL_LightShowStopReq_flg
  slr_VHAL_MFRDNBrightReq_pct : BusSelector  OutputSignals=VHAL_MFRDNBrightReq_pct
  slr_VHAL_OFFACMODE_enum : BusSelector  OutputSignals=VHAL_OFFACMODE_enum
  slr_VHAL_PSEATventreq_enum : BusSelector  OutputSignals=VHAL_PSEATventreq_enum
  slr_VHAL_PerdV2L_enum : BusSelector  OutputSignals=VHAL_PerdV2L_enum
  slr_VHAL_RFogLampSW_flg : BusSelector  OutputSignals=VHAL_RFogLampSW_flg
  slr_VHAL_RollModeSWCmd_enum : BusSelector  OutputSignals=VHAL_RollModeSWCmd_enum
  slr_VHAL_RoomLampMode_flg : BusSelector  OutputSignals=VHAL_RoomLampMode_flg
  slr_VHAL_SOCADJBUTT_flg : BusSelector  OutputSignals=VHAL_SOCADJBUTT_flg
  slr_VHAL_SOCLimitSet_pct : BusSelector  OutputSignals=VHAL_SOCLimitSet_pct
  slr_VHAL_SOCV2LLimit_pct : BusSelector  OutputSignals=VHAL_SOCV2LLimit_pct
  slr_VHAL_SchedChgStart_flg : BusSelector  OutputSignals=VHAL_SchedChgStart_flg
  slr_VHAL_SchedChgStop_flg : BusSelector  OutputSignals=VHAL_SchedChgStop_flg
  slr_VHAL_SchedChgbutt_flg : BusSelector  OutputSignals=VHAL_SchedChgbutt_flg
  slr_VHAL_SchedChglimit_pct : BusSelector  OutputSignals=VHAL_SchedChglimit_pct
  slr_VHAL_SchedChgwake_flg : BusSelector  OutputSignals=VHAL_SchedChgwake_flg
  slr_VHAL_SenstivityPosition_enum : BusSelector  OutputSignals=VHAL_SenstivityPosition_enum
  slr_VHAL_SetUnlockSingle_flg : BusSelector  OutputSignals=VHAL_SetUnlockSingle_flg
  slr_VHAL_TCSSWCmd_enum : BusSelector  OutputSignals=VHAL_TCSSWCmd_enum
  slr_VHAL_TPMSCaliButt_flg : BusSelector  OutputSignals=VHAL_TPMSCaliButt_flg
  slr_VHAL_TPMSResButt_flg : BusSelector  OutputSignals=VHAL_TPMSResButt_flg
  slr_VHAL_TurnSwTimeSet_enum : BusSelector  OutputSignals=VHAL_TurnSwTimeSet_enum
  slr_VHAL_WalkawayLockSW_flg : BusSelector  OutputSignals=VHAL_WalkawayLockSW_flg
  slr_VHAL_WlcmLightMode_enum : BusSelector  OutputSignals=VHAL_WlcmLightMode_enum
  slr_VHAL_sigAirIntenZon1Req_enum : BusSelector  OutputSignals=VHAL_sigAirIntenZon1Req_enum
  slr_VHAL_sigDfrstReq_flg : BusSelector  OutputSignals=VHAL_sigDfrstReq_flg
  slr_VHAL_sigFaceReq_flg : BusSelector  OutputSignals=VHAL_sigFaceReq_flg
  slr_VHAL_sigFootReq_flg : BusSelector  OutputSignals=VHAL_sigFootReq_flg
  slr_VHAL_sigRecircReq_flg : BusSelector  OutputSignals=VHAL_sigRecircReq_flg
  slr_VHAL_sigSetTempZon1Req_C : BusSelector  OutputSignals=VHAL_sigSetTempZon1Req_C
  slr_VHAL_sigSetTempZon2Req_C : BusSelector  OutputSignals=VHAL_sigSetTempZon2Req_C
  VINP_ACChgCurSet_A : Outport
  VINP_AVMErrSTA_flg : Outport  Port=2
  VINP_AVMOFFRecButt_flg : Outport  Port=3
  VINP_AVMParkingmode_enum : Outport  Port=4
  VINP_AVMparkingcancel_enum : Outport  Port=5
  VINP_AVMparkingexcute_enum : Outport  Port=6
  VINP_CAASSw_enum : Outport  Port=7
  VINP_CDLLockButt_flg : Outport  Port=8
  VINP_CDLUnlockButt_flg : Outport  Port=9
  VINP_DSEATantiset_flg : Outport  Port=10
  VINP_DSEATentryfunset_flg : Outport  Port=11
  VINP_DSEATventreq_enum : Outport  Port=12
  VINP_Distanceunit_flg : Outport  Port=13
  VINP_ESCSWCmd_enum : Outport  Port=14
  VINP_FSOffSw_enum : Outport  Port=15
  VINP_FollowMeSW_flg : Outport  Port=16
  VINP_GPSLAT_s : Outport  Port=17
  VINP_GPSLONG_enum : Outport  Port=18
  VINP_HeadLampSW_enum : Outport  Port=19
  VINP_HoodLatchSW_enum : Outport  Port=20
  VINP_IVINightModeSta_flg : Outport  Port=21
  VINP_IVIPTGModeSW_enum : Outport  Port=22
  VINP_IVIPTGStaSW_enum : Outport  Port=23
  VINP_IVIPTGUSStaSW_flg : Outport  Port=24
  VINP_IVIPWModeReq_enum : Outport  Port=25
  VINP_IVIPwrLockSW_enum : Outport  Port=26
  VINP_IVIPwroffreq_flg : Outport  Port=27
  VINP_IVIRRDefReq_flg : Outport  Port=28
  VINP_IVIReqV2L_enum : Outport  Port=29
  VINP_IVIScreen_enum : Outport  Port=30
  VINP_IVIStartChgreq_flg : Outport  Port=31
  VINP_IVIStatus_flg : Outport  Port=32
  VINP_IVIStopChgreq_flg : Outport  Port=33
  VINP_IVITriggerreq_flg : Outport  Port=34
  VINP_IVIUnlockChgreq_flg : Outport  Port=35
  VINP_IVIWIMAINSW_flg : Outport  Port=36
  VINP_LDrvControlCommand_pct : Outport  Port=37
  VINP_LPasControlCommand_pct : Outport  Port=38
  VINP_LRLDControlCommand_pct : Outport  Port=39
  VINP_LRRDControlCommand_pct : Outport  Port=40
  VINP_LightShowStartReq_flg : Outport  Port=41
  VINP_LightShowStopReq_flg : Outport  Port=42
  VINP_MFRDNBrightReq_pct : Outport  Port=43
  VINP_OFFACMODE_enum : Outport  Port=44
  VINP_PSEATventreq_enum : Outport  Port=45
  VINP_PerdV2L_enum : Outport  Port=46
  VINP_RFogLampSW_flg : Outport  Port=47
  VINP_RollModeSWCmd_enum : Outport  Port=48
  VINP_RoomLampMode_flg : Outport  Port=49
  VINP_SOCADJBUTT_flg : Outport  Port=50
  VINP_SOCLimitSet_pct : Outport  Port=51
  VINP_SOCV2LLimit_pct : Outport  Port=52
  VINP_SchedChgStart_flg : Outport  Port=53
  VINP_SchedChgStop_flg : Outport  Port=54
  VINP_SchedChgbutt_flg : Outport  Port=55
  VINP_SchedChglimit_pct : Outport  Port=56
  VINP_SchedChgwake_flg : Outport  Port=57
  VINP_SenstivityPosition_enum : Outport  Port=58
  VINP_SetUnlockSingle_flg : Outport  Port=59
  VINP_TCSSWCmd_enum : Outport  Port=60
  VINP_TPMSCaliButt_flg : Outport  Port=61
  VINP_TPMSResButt_flg : Outport  Port=62
  VINP_TurnSwTimeSet_enum : Outport  Port=63
  VINP_WalkawayLockSW_flg : Outport  Port=64
  VINP_WlcmLightMode_enum : Outport  Port=65
  VINP_sigAirIntenZon1Req_enum : Outport  Port=66
  VINP_sigDfrstReq_flg : Outport  Port=67
  VINP_sigFaceReq_flg : Outport  Port=68
  VINP_sigFootReq_flg : Outport  Port=69
  VINP_sigRecircReq_flg : Outport  Port=70
  VINP_sigSetTempZon1Req_C : Outport  Port=71
  VINP_sigSetTempZon2Req_C : Outport  Port=72
  wires:
  BHAL_outputs/1 -> [BHAL_outputs]
  inp_CanValid_bus/1 -> [inp_CanValid_bus]
  [BHAL_outputs] -> slr_VHAL_ACChgCurSet_A/1
  slr_VHAL_ACChgCurSet_A/1 -> ACChgCurSet/1  "<VHAL_ACChgCurSet_A>"
  True_VHAL_ACChgCurSet_A/1 -> ACChgCurSet/2
  [inp_CanValid_bus] -> slr1_1/1
  slr1_1/1 -> ACChgCurSet/3  "<VINP_CANMsgValidIVI2_flg>"
  ACChgCurSet/1 -> VINP_ACChgCurSet_A/1  "VINP_ACChgCurSet_A"
  ACChgCurSet/2 -> Terminator_1/1
  [BHAL_outputs] -> slr_VHAL_AVMErrSTA_flg/1
  slr_VHAL_AVMErrSTA_flg/1 -> AVMErrSTA/1  "<VHAL_AVMErrSTA_flg>"
  True_VHAL_AVMErrSTA_flg/1 -> AVMErrSTA/2
  [inp_CanValid_bus] -> slr1_2/1
  slr1_2/1 -> AVMErrSTA/3  "<VINP_CANMsgValidIVI2_flg>"
  AVMErrSTA/1 -> VINP_AVMErrSTA_flg/1  "VINP_AVMErrSTA_flg"
  AVMErrSTA/2 -> Terminator_2/1
  [BHAL_outputs] -> slr_VHAL_AVMOFFRecButt_flg/1
  slr_VHAL_AVMOFFRecButt_flg/1 -> AVMOFFRecButt/1  "<VHAL_AVMOFFRecButt_flg>"
  True_VHAL_AVMOFFRecButt_flg/1 -> AVMOFFRecButt/2
  [inp_CanValid_bus] -> slr1_3/1
  slr1_3/1 -> AVMOFFRecButt/3  "<VINP_CANMsgValidIVI2_flg>"
  AVMOFFRecButt/1 -> VINP_AVMOFFRecButt_flg/1  "VINP_AVMOFFRecButt_flg"
  AVMOFFRecButt/2 -> Terminator_3/1
  [BHAL_outputs] -> slr_VHAL_AVMParkingmode_enum/1
  slr_VHAL_AVMParkingmode_enum/1 -> AVMParkingmode/1  "<VHAL_AVMParkingmode_enum>"
  True_VHAL_AVMParkingmode_enum/1 -> AVMParkingmode/2
  [inp_CanValid_bus] -> slr1_4/1
  slr1_4/1 -> AVMParkingmode/3  "<VINP_CANMsgValidIVI2_flg>"
  AVMParkingmode/1 -> VINP_AVMParkingmode_enum/1  "VINP_AVMParkingmode_enum"
  AVMParkingmode/2 -> Terminator_4/1
  [BHAL_outputs] -> slr_VHAL_AVMparkingcancel_enum/1
  slr_VHAL_AVMparkingcancel_enum/1 -> AVMparkingcancel/1  "<VHAL_AVMparkingcancel_enum>"
  True_VHAL_AVMparkingcancel_enum/1 -> AVMparkingcancel/2
  [inp_CanValid_bus] -> slr1_5/1
  slr1_5/1 -> AVMparkingcancel/3  "<VINP_CANMsgValidIVI2_flg>"
  AVMparkingcancel/1 -> VINP_AVMparkingcancel_enum/1  "VINP_AVMparkingcancel_enum"
  AVMparkingcancel/2 -> Terminator_5/1
  [BHAL_outputs] -> slr_VHAL_AVMparkingexcute_enum/1
  slr_VHAL_AVMparkingexcute_enum/1 -> AVMparkingexcute/1  "<VHAL_AVMparkingexcute_enum>"
  True_VHAL_AVMparkingexcute_enum/1 -> AVMparkingexcute/2
  [inp_CanValid_bus] -> slr1_6/1
  slr1_6/1 -> AVMparkingexcute/3  "<VINP_CANMsgValidIVI2_flg>"
  AVMparkingexcute/1 -> VINP_AVMparkingexcute_enum/1  "VINP_AVMparkingexcute_enum"
  AVMparkingexcute/2 -> Terminator_6/1
  [BHAL_outputs] -> slr_VHAL_CAASSw_enum/1
  slr_VHAL_CAASSw_enum/1 -> CAASSw/1  "<VHAL_CAASSw_enum>"
  True_VHAL_CAASSw_enum/1 -> CAASSw/2
  [inp_CanValid_bus] -> slr1_7/1
  slr1_7/1 -> CAASSw/3  "<VINP_CANMsgValidIVI2_flg>"
  CAASSw/1 -> VINP_CAASSw_enum/1  "VINP_CAASSw_enum"
  CAASSw/2 -> Terminator_7/1
  [BHAL_outputs] -> slr_VHAL_CDLLockButt_flg/1
  slr_VHAL_CDLLockButt_flg/1 -> CDLLockButt/1  "<VHAL_CDLLockButt_flg>"
  True_VHAL_CDLLockButt_flg/1 -> CDLLockButt/2
  [inp_CanValid_bus] -> slr1_8/1
  slr1_8/1 -> CDLLockButt/3  "<VINP_CANMsgValidIVI2_flg>"
  CDLLockButt/1 -> VINP_CDLLockButt_flg/1  "VINP_CDLLockButt_flg"
  CDLLockButt/2 -> Terminator_8/1
  [BHAL_outputs] -> slr_VHAL_CDLUnlockButt_flg/1
  slr_VHAL_CDLUnlockButt_flg/1 -> CDLUnlockButt/1  "<VHAL_CDLUnlockButt_flg>"
  True_VHAL_CDLUnlockButt_flg/1 -> CDLUnlockButt/2
  [inp_CanValid_bus] -> slr1_9/1
  slr1_9/1 -> CDLUnlockButt/3  "<VINP_CANMsgValidIVI2_flg>"
  CDLUnlockButt/1 -> VINP_CDLUnlockButt_flg/1  "VINP_CDLUnlockButt_flg"
  CDLUnlockButt/2 -> Terminator_9/1
  [BHAL_outputs] -> slr_VHAL_DSEATantiset_flg/1
  slr_VHAL_DSEATantiset_flg/1 -> DSEATantiset/1  "<VHAL_DSEATantiset_flg>"
  True_VHAL_DSEATantiset_flg/1 -> DSEATantiset/2
  [inp_CanValid_bus] -> slr1_10/1
  slr1_10/1 -> DSEATantiset/3  "<VINP_CANMsgValidIVI2_flg>"
  DSEATantiset/1 -> VINP_DSEATantiset_flg/1  "VINP_DSEATantiset_flg"
  DSEATantiset/2 -> Terminator_10/1
  [BHAL_outputs] -> slr_VHAL_DSEATentryfunset_flg/1
  slr_VHAL_DSEATentryfunset_flg/1 -> DSEATentryfunset/1  "<VHAL_DSEATentryfunset_flg>"
  True_VHAL_DSEATentryfunset_flg/1 -> DSEATentryfunset/2
  [inp_CanValid_bus] -> slr1_11/1
  slr1_11/1 -> DSEATentryfunset/3  "<VINP_CANMsgValidIVI2_flg>"
  DSEATentryfunset/1 -> VINP_DSEATentryfunset_flg/1  "VINP_DSEATentryfunset_flg"
  DSEATentryfunset/2 -> Terminator_11/1
  [BHAL_outputs] -> slr_VHAL_DSEATventreq_enum/1
  slr_VHAL_DSEATventreq_enum/1 -> DSEATventreq/1  "<VHAL_DSEATventreq_enum>"
  True_VHAL_DSEATventreq_enum/1 -> DSEATventreq/2
  [inp_CanValid_bus] -> slr1_12/1
  slr1_12/1 -> DSEATventreq/3  "<VINP_CANMsgValidIVI2_flg>"
  DSEATventreq/1 -> VINP_DSEATventreq_enum/1  "VINP_DSEATventreq_enum"
  DSEATventreq/2 -> Terminator_12/1
  [BHAL_outputs] -> slr_VHAL_Distanceunit_flg/1
  slr_VHAL_Distanceunit_flg/1 -> Distanceunit/1  "<VHAL_Distanceunit_flg>"
  True_VHAL_Distanceunit_flg/1 -> Distanceunit/2
  [inp_CanValid_bus] -> slr1_13/1
  slr1_13/1 -> Distanceunit/3  "<VINP_CANMsgValidIVI2_flg>"
  Distanceunit/1 -> VINP_Distanceunit_flg/1  "VINP_Distanceunit_flg"
  Distanceunit/2 -> Terminator_13/1
  [BHAL_outputs] -> slr_VHAL_ESCSWCmd_enum/1
  slr_VHAL_ESCSWCmd_enum/1 -> ESCSWCmd/1  "<VHAL_ESCSWCmd_enum>"
  True_VHAL_ESCSWCmd_enum/1 -> ESCSWCmd/2
  [inp_CanValid_bus] -> slr1_14/1
  slr1_14/1 -> ESCSWCmd/3  "<VINP_CANMsgValidIVI2_flg>"
  ESCSWCmd/1 -> VINP_ESCSWCmd_enum/1  "VINP_ESCSWCmd_enum"
  ESCSWCmd/2 -> Terminator_14/1
  [BHAL_outputs] -> slr_VHAL_FSOffSw_enum/1
  slr_VHAL_FSOffSw_enum/1 -> FSOffSw/1  "<VHAL_FSOffSw_enum>"
  True_VHAL_FSOffSw_enum/1 -> FSOffSw/2
  [inp_CanValid_bus] -> slr1_15/1
  slr1_15/1 -> FSOffSw/3  "<VINP_CANMsgValidIVI2_flg>"
  FSOffSw/1 -> VINP_FSOffSw_enum/1  "VINP_FSOffSw_enum"
  FSOffSw/2 -> Terminator_15/1
  [BHAL_outputs] -> slr_VHAL_FollowMeSW_flg/1
  slr_VHAL_FollowMeSW_flg/1 -> FollowMeSW/1  "<VHAL_FollowMeSW_flg>"
  True_VHAL_FollowMeSW_flg/1 -> FollowMeSW/2
  [inp_CanValid_bus] -> slr1_16/1
  slr1_16/1 -> FollowMeSW/3  "<VINP_CANMsgValidIVI2_flg>"
  FollowMeSW/1 -> VINP_FollowMeSW_flg/1  "VINP_FollowMeSW_flg"
  FollowMeSW/2 -> Terminator_16/1
  [BHAL_outputs] -> slr_VHAL_GPSLAT_s/1
  slr_VHAL_GPSLAT_s/1 -> GPSLAT/1  "<VHAL_GPSLAT_s>"
  True_VHAL_GPSLAT_s/1 -> GPSLAT/2
  [inp_CanValid_bus] -> slr1_17/1
  slr1_17/1 -> GPSLAT/3  "<VINP_CANMsgValidIVI2_flg>"
  GPSLAT/1 -> VINP_GPSLAT_s/1  "VINP_GPSLAT_s"
  GPSLAT/2 -> Terminator_17/1
  [BHAL_outputs] -> slr_VHAL_GPSLONG_enum/1
  slr_VHAL_GPSLONG_enum/1 -> GPSLONG/1  "<VHAL_GPSLONG_enum>"
  True_VHAL_GPSLONG_enum/1 -> GPSLONG/2
  [inp_CanValid_bus] -> slr1_18/1
  slr1_18/1 -> GPSLONG/3  "<VINP_CANMsgValidIVI2_flg>"
  GPSLONG/1 -> VINP_GPSLONG_enum/1  "VINP_GPSLONG_enum"
  GPSLONG/2 -> Terminator_18/1
  [BHAL_outputs] -> slr_VHAL_HeadLampSW_enum/1
  slr_VHAL_HeadLampSW_enum/1 -> HeadLampSW/1  "<VHAL_HeadLampSW_enum>"
  True_VHAL_HeadLampSW_enum/1 -> HeadLampSW/2
  [inp_CanValid_bus] -> slr1_19/1
  slr1_19/1 -> HeadLampSW/3  "<VINP_CANMsgValidIVI2_flg>"
  HeadLampSW/1 -> VINP_HeadLampSW_enum/1  "VINP_HeadLampSW_enum"
  HeadLampSW/2 -> Terminator_19/1
  [BHAL_outputs] -> slr_VHAL_HoodLatchSW_enum/1
  slr_VHAL_HoodLatchSW_enum/1 -> HoodLatchSW/1  "<VHAL_HoodLatchSW_enum>"
  True_VHAL_HoodLatchSW_enum/1 -> HoodLatchSW/2
  [inp_CanValid_bus] -> slr1_20/1
  slr1_20/1 -> HoodLatchSW/3  "<VINP_CANMsgValidIVI2_flg>"
  HoodLatchSW/1 -> VINP_HoodLatchSW_enum/1  "VINP_HoodLatchSW_enum"
  HoodLatchSW/2 -> Terminator_20/1
  [BHAL_outputs] -> slr_VHAL_IVINightModeSta_flg/1
  slr_VHAL_IVINightModeSta_flg/1 -> IVINightModeSta/1  "<VHAL_IVINightModeSta_flg>"
  True_VHAL_IVINightModeSta_flg/1 -> IVINightModeSta/2
  [inp_CanValid_bus] -> slr1_21/1
  slr1_21/1 -> IVINightModeSta/3  "<VINP_CANMsgValidIVI2_flg>"
  IVINightModeSta/1 -> VINP_IVINightModeSta_flg/1  "VINP_IVINightModeSta_flg"
  IVINightModeSta/2 -> Terminator_21/1
  [BHAL_outputs] -> slr_VHAL_IVIPTGModeSW_enum/1
  slr_VHAL_IVIPTGModeSW_enum/1 -> IVIPTGModeSW/1  "<VHAL_IVIPTGModeSW_enum>"
  True_VHAL_IVIPTGModeSW_enum/1 -> IVIPTGModeSW/2
  [inp_CanValid_bus] -> slr1_22/1
  slr1_22/1 -> IVIPTGModeSW/3  "<VINP_CANMsgValidIVI2_flg>"
  IVIPTGModeSW/1 -> VINP_IVIPTGModeSW_enum/1  "VINP_IVIPTGModeSW_enum"
  IVIPTGModeSW/2 -> Terminator_22/1
  [BHAL_outputs] -> slr_VHAL_IVIPTGStaSW_enum/1
  slr_VHAL_IVIPTGStaSW_enum/1 -> IVIPTGStaSW/1  "<VHAL_IVIPTGStaSW_enum>"
  True_VHAL_IVIPTGStaSW_enum/1 -> IVIPTGStaSW/2
  [inp_CanValid_bus] -> slr1_23/1
  slr1_23/1 -> IVIPTGStaSW/3  "<VINP_CANMsgValidIVI2_flg>"
  IVIPTGStaSW/1 -> VINP_IVIPTGStaSW_enum/1  "VINP_IVIPTGStaSW_enum"
  IVIPTGStaSW/2 -> Terminator_23/1
  [BHAL_outputs] -> slr_VHAL_IVIPTGUSStaSW_flg/1
  slr_VHAL_IVIPTGUSStaSW_flg/1 -> IVIPTGUSStaSW/1  "<VHAL_IVIPTGUSStaSW_flg>"
  True_VHAL_IVIPTGUSStaSW_flg/1 -> IVIPTGUSStaSW/2
  [inp_CanValid_bus] -> slr1_24/1
  slr1_24/1 -> IVIPTGUSStaSW/3  "<VINP_CANMsgValidIVI2_flg>"
  IVIPTGUSStaSW/1 -> VINP_IVIPTGUSStaSW_flg/1  "VINP_IVIPTGUSStaSW_flg"
  IVIPTGUSStaSW/2 -> Terminator_24/1
  [BHAL_outputs] -> slr_VHAL_IVIPWModeReq_enum/1
  slr_VHAL_IVIPWModeReq_enum/1 -> IVIPWModeReq/1  "<VHAL_IVIPWModeReq_enum>"
  True_VHAL_IVIPWModeReq_enum/1 -> IVIPWModeReq/2
  [inp_CanValid_bus] -> slr1_25/1
  slr1_25/1 -> IVIPWModeReq/3  "<VINP_CANMsgValidIVI2_flg>"
  IVIPWModeReq/1 -> VINP_IVIPWModeReq_enum/1  "VINP_IVIPWModeReq_enum"
  IVIPWModeReq/2 -> Terminator_25/1
  [BHAL_outputs] -> slr_VHAL_IVIPwrLockSW_enum/1
  slr_VHAL_IVIPwrLockSW_enum/1 -> IVIPwrLockSW/1  "<VHAL_IVIPwrLockSW_enum>"
  True_VHAL_IVIPwrLockSW_enum/1 -> IVIPwrLockSW/2
  [inp_CanValid_bus] -> slr1_26/1
  slr1_26/1 -> IVIPwrLockSW/3  "<VINP_CANMsgValidIVI2_flg>"
  IVIPwrLockSW/1 -> VINP_IVIPwrLockSW_enum/1  "VINP_IVIPwrLockSW_enum"
  IVIPwrLockSW/2 -> Terminator_26/1
  [BHAL_outputs] -> slr_VHAL_IVIPwroffreq_flg/1
  slr_VHAL_IVIPwroffreq_flg/1 -> IVIPwroffreq/1  "<VHAL_IVIPwroffreq_flg>"
  True_VHAL_IVIPwroffreq_flg/1 -> IVIPwroffreq/2
  [inp_CanValid_bus] -> slr1_27/1
  slr1_27/1 -> IVIPwroffreq/3  "<VINP_CANMsgValidIVI2_flg>"
  IVIPwroffreq/1 -> VINP_IVIPwroffreq_flg/1  "VINP_IVIPwroffreq_flg"
  IVIPwroffreq/2 -> Terminator_27/1
  [BHAL_outputs] -> slr_VHAL_IVIRRDefReq_flg/1
  slr_VHAL_IVIRRDefReq_flg/1 -> IVIRRDefReq/1  "<VHAL_IVIRRDefReq_flg>"
  True_VHAL_IVIRRDefReq_flg/1 -> IVIRRDefReq/2
  [inp_CanValid_bus] -> slr1_28/1
  slr1_28/1 -> IVIRRDefReq/3  "<VINP_CANMsgValidIVI2_flg>"
  IVIRRDefReq/1 -> VINP_IVIRRDefReq_flg/1  "VINP_IVIRRDefReq_flg"
  IVIRRDefReq/2 -> Terminator_28/1
  [BHAL_outputs] -> slr_VHAL_IVIReqV2L_enum/1
  slr_VHAL_IVIReqV2L_enum/1 -> IVIReqV2L/1  "<VHAL_IVIReqV2L_enum>"
  True_VHAL_IVIReqV2L_enum/1 -> IVIReqV2L/2
  [inp_CanValid_bus] -> slr1_29/1
  slr1_29/1 -> IVIReqV2L/3  "<VINP_CANMsgValidIVI2_flg>"
  IVIReqV2L/1 -> VINP_IVIReqV2L_enum/1  "VINP_IVIReqV2L_enum"
  IVIReqV2L/2 -> Terminator_29/1
  [BHAL_outputs] -> slr_VHAL_IVIScreen_enum/1
  slr_VHAL_IVIScreen_enum/1 -> IVIScreen/1  "<VHAL_IVIScreen_enum>"
  True_VHAL_IVIScreen_enum/1 -> IVIScreen/2
  [inp_CanValid_bus] -> slr1_30/1
  slr1_30/1 -> IVIScreen/3  "<VINP_CANMsgValidIVI2_flg>"
  IVIScreen/1 -> VINP_IVIScreen_enum/1  "VINP_IVIScreen_enum"
  IVIScreen/2 -> Terminator_30/1
  [BHAL_outputs] -> slr_VHAL_IVIStartChgreq_flg/1
  slr_VHAL_IVIStartChgreq_flg/1 -> IVIStartChgreq/1  "<VHAL_IVIStartChgreq_flg>"
  True_VHAL_IVIStartChgreq_flg/1 -> IVIStartChgreq/2
  [inp_CanValid_bus] -> slr1_31/1
  slr1_31/1 -> IVIStartChgreq/3  "<VINP_CANMsgValidIVI2_flg>"
  IVIStartChgreq/1 -> VINP_IVIStartChgreq_flg/1  "VINP_IVIStartChgreq_flg"
  IVIStartChgreq/2 -> Terminator_31/1
  [BHAL_outputs] -> slr_VHAL_IVIStatus_flg/1
  slr_VHAL_IVIStatus_flg/1 -> IVIStatus/1  "<VHAL_IVIStatus_flg>"
  True_VHAL_IVIStatus_flg/1 -> IVIStatus/2
  [inp_CanValid_bus] -> slr1_32/1
  slr1_32/1 -> IVIStatus/3  "<VINP_CANMsgValidIVI2_flg>"
  IVIStatus/1 -> VINP_IVIStatus_flg/1  "VINP_IVIStatus_flg"
  IVIStatus/2 -> Terminator_32/1
  [BHAL_outputs] -> slr_VHAL_IVIStopChgreq_flg/1
  slr_VHAL_IVIStopChgreq_flg/1 -> IVIStopChgreq/1  "<VHAL_IVIStopChgreq_flg>"
  True_VHAL_IVIStopChgreq_flg/1 -> IVIStopChgreq/2
  [inp_CanValid_bus] -> slr1_33/1
  slr1_33/1 -> IVIStopChgreq/3  "<VINP_CANMsgValidIVI2_flg>"
  IVIStopChgreq/1 -> VINP_IVIStopChgreq_flg/1  "VINP_IVIStopChgreq_flg"
  IVIStopChgreq/2 -> Terminator_33/1
  [BHAL_outputs] -> slr_VHAL_IVITriggerreq_flg/1
  slr_VHAL_IVITriggerreq_flg/1 -> IVITriggerreq/1  "<VHAL_IVITriggerreq_flg>"
  True_VHAL_IVITriggerreq_flg/1 -> IVITriggerreq/2
  [inp_CanValid_bus] -> slr1_34/1
  slr1_34/1 -> IVITriggerreq/3  "<VINP_CANMsgValidIVI2_flg>"
  IVITriggerreq/1 -> VINP_IVITriggerreq_flg/1  "VINP_IVITriggerreq_flg"
  IVITriggerreq/2 -> Terminator_34/1
  [BHAL_outputs] -> slr_VHAL_IVIUnlockChgreq_flg/1
  slr_VHAL_IVIUnlockChgreq_flg/1 -> IVIUnlockChgreq/1  "<VHAL_IVIUnlockChgreq_flg>"
  True_VHAL_IVIUnlockChgreq_flg/1 -> IVIUnlockChgreq/2
  [inp_CanValid_bus] -> slr1_35/1
  slr1_35/1 -> IVIUnlockChgreq/3  "<VINP_CANMsgValidIVI2_flg>"
  IVIUnlockChgreq/1 -> VINP_IVIUnlockChgreq_flg/1  "VINP_IVIUnlockChgreq_flg"
  IVIUnlockChgreq/2 -> Terminator_35/1
  [BHAL_outputs] -> slr_VHAL_IVIWIMAINSW_flg/1
  slr_VHAL_IVIWIMAINSW_flg/1 -> IVIWIMAINSW/1  "<VHAL_IVIWIMAINSW_flg>"
  True_VHAL_IVIWIMAINSW_flg/1 -> IVIWIMAINSW/2
  [inp_CanValid_bus] -> slr1_36/1
  slr1_36/1 -> IVIWIMAINSW/3  "<VINP_CANMsgValidIVI2_flg>"
  IVIWIMAINSW/1 -> VINP_IVIWIMAINSW_flg/1  "VINP_IVIWIMAINSW_flg"
  IVIWIMAINSW/2 -> Terminator_36/1
  [BHAL_outputs] -> slr_VHAL_LDrvControlCommand_pct/1
  slr_VHAL_LDrvControlCommand_pct/1 -> LDrvControlCommand/1  "<VHAL_LDrvControlCommand_pct>"
  True_VHAL_LDrvControlCommand_pct/1 -> LDrvControlCommand/2
  [inp_CanValid_bus] -> slr1_37/1
  slr1_37/1 -> LDrvControlCommand/3  "<VINP_CANMsgValidIVI2_flg>"
  LDrvControlCommand/1 -> VINP_LDrvControlCommand_pct/1  "VINP_LDrvControlCommand_pct"
  LDrvControlCommand/2 -> Terminator_37/1
  [BHAL_outputs] -> slr_VHAL_LPasControlCommand_pct/1
  slr_VHAL_LPasControlCommand_pct/1 -> LPasControlCommand/1  "<VHAL_LPasControlCommand_pct>"
  True_VHAL_LPasControlCommand_pct/1 -> LPasControlCommand/2
  [inp_CanValid_bus] -> slr1_38/1
  slr1_38/1 -> LPasControlCommand/3  "<VINP_CANMsgValidIVI2_flg>"
  LPasControlCommand/1 -> VINP_LPasControlCommand_pct/1  "VINP_LPasControlCommand_pct"
  LPasControlCommand/2 -> Terminator_38/1
  [BHAL_outputs] -> slr_VHAL_LRLDControlCommand_pct/1
  slr_VHAL_LRLDControlCommand_pct/1 -> LRLDControlCommand/1  "<VHAL_LRLDControlCommand_pct>"
  True_VHAL_LRLDControlCommand_pct/1 -> LRLDControlCommand/2
  [inp_CanValid_bus] -> slr1_39/1
  slr1_39/1 -> LRLDControlCommand/3  "<VINP_CANMsgValidIVI2_flg>"
  LRLDControlCommand/1 -> VINP_LRLDControlCommand_pct/1  "VINP_LRLDControlCommand_pct"
  LRLDControlCommand/2 -> Terminator_39/1
  [BHAL_outputs] -> slr_VHAL_LRRDControlCommand_pct/1
  slr_VHAL_LRRDControlCommand_pct/1 -> LRRDControlCommand/1  "<VHAL_LRRDControlCommand_pct>"
  True_VHAL_LRRDControlCommand_pct/1 -> LRRDControlCommand/2
  [inp_CanValid_bus] -> slr1_40/1
  slr1_40/1 -> LRRDControlCommand/3  "<VINP_CANMsgValidIVI2_flg>"
  LRRDControlCommand/1 -> VINP_LRRDControlCommand_pct/1  "VINP_LRRDControlCommand_pct"
  LRRDControlCommand/2 -> Terminator_40/1
  [BHAL_outputs] -> slr_VHAL_LightShowStartReq_flg/1
  slr_VHAL_LightShowStartReq_flg/1 -> LightShowStartReq/1  "<VHAL_LightShowStartReq_flg>"
  True_VHAL_LightShowStartReq_flg/1 -> LightShowStartReq/2
  [inp_CanValid_bus] -> slr1_41/1
  slr1_41/1 -> LightShowStartReq/3  "<VINP_CANMsgValidIVI2_flg>"
  LightShowStartReq/1 -> VINP_LightShowStartReq_flg/1  "VINP_LightShowStartReq_flg"
  LightShowStartReq/2 -> Terminator_41/1
  [BHAL_outputs] -> slr_VHAL_LightShowStopReq_flg/1
  slr_VHAL_LightShowStopReq_flg/1 -> LightShowStopReq/1  "<VHAL_LightShowStopReq_flg>"
  True_VHAL_LightShowStopReq_flg/1 -> LightShowStopReq/2
  [inp_CanValid_bus] -> slr1_42/1
  slr1_42/1 -> LightShowStopReq/3  "<VINP_CANMsgValidIVI2_flg>"
  LightShowStopReq/1 -> VINP_LightShowStopReq_flg/1  "VINP_LightShowStopReq_flg"
  LightShowStopReq/2 -> Terminator_42/1
  [BHAL_outputs] -> slr_VHAL_MFRDNBrightReq_pct/1
  slr_VHAL_MFRDNBrightReq_pct/1 -> MFRDNBrightReq/1  "<VHAL_MFRDNBrightReq_pct>"
  True_VHAL_MFRDNBrightReq_pct/1 -> MFRDNBrightReq/2
  [inp_CanValid_bus] -> slr1_43/1
  slr1_43/1 -> MFRDNBrightReq/3  "<VINP_CANMsgValidIVI2_flg>"
  MFRDNBrightReq/1 -> VINP_MFRDNBrightReq_pct/1  "VINP_MFRDNBrightReq_pct"
  MFRDNBrightReq/2 -> Terminator_43/1
  [BHAL_outputs] -> slr_VHAL_OFFACMODE_enum/1
  slr_VHAL_OFFACMODE_enum/1 -> OFFACMODE/1  "<VHAL_OFFACMODE_enum>"
  True_VHAL_OFFACMODE_enum/1 -> OFFACMODE/2
  [inp_CanValid_bus] -> slr1_44/1
  slr1_44/1 -> OFFACMODE/3  "<VINP_CANMsgValidIVI2_flg>"
  OFFACMODE/1 -> VINP_OFFACMODE_enum/1  "VINP_OFFACMODE_enum"
  OFFACMODE/2 -> Terminator_44/1
  [BHAL_outputs] -> slr_VHAL_PSEATventreq_enum/1
  slr_VHAL_PSEATventreq_enum/1 -> PSEATventreq/1  "<VHAL_PSEATventreq_enum>"
  True_VHAL_PSEATventreq_enum/1 -> PSEATventreq/2
  [inp_CanValid_bus] -> slr1_45/1
  slr1_45/1 -> PSEATventreq/3  "<VINP_CANMsgValidIVI2_flg>"
  PSEATventreq/1 -> VINP_PSEATventreq_enum/1  "VINP_PSEATventreq_enum"
  PSEATventreq/2 -> Terminator_45/1
  [BHAL_outputs] -> slr_VHAL_PerdV2L_enum/1
  slr_VHAL_PerdV2L_enum/1 -> PerdV2L/1  "<VHAL_PerdV2L_enum>"
  True_VHAL_PerdV2L_enum/1 -> PerdV2L/2
  [inp_CanValid_bus] -> slr1_46/1
  slr1_46/1 -> PerdV2L/3  "<VINP_CANMsgValidIVI2_flg>"
  PerdV2L/1 -> VINP_PerdV2L_enum/1  "VINP_PerdV2L_enum"
  PerdV2L/2 -> Terminator_46/1
  [BHAL_outputs] -> slr_VHAL_RFogLampSW_flg/1
  slr_VHAL_RFogLampSW_flg/1 -> RFogLampSW/1  "<VHAL_RFogLampSW_flg>"
  True_VHAL_RFogLampSW_flg/1 -> RFogLampSW/2
  [inp_CanValid_bus] -> slr1_47/1
  slr1_47/1 -> RFogLampSW/3  "<VINP_CANMsgValidIVI2_flg>"
  RFogLampSW/1 -> VINP_RFogLampSW_flg/1  "VINP_RFogLampSW_flg"
  RFogLampSW/2 -> Terminator_47/1
  [BHAL_outputs] -> slr_VHAL_RollModeSWCmd_enum/1
  slr_VHAL_RollModeSWCmd_enum/1 -> RollModeSWCmd/1  "<VHAL_RollModeSWCmd_enum>"
  True_VHAL_RollModeSWCmd_enum/1 -> RollModeSWCmd/2
  [inp_CanValid_bus] -> slr1_48/1
  slr1_48/1 -> RollModeSWCmd/3  "<VINP_CANMsgValidIVI2_flg>"
  RollModeSWCmd/1 -> VINP_RollModeSWCmd_enum/1  "VINP_RollModeSWCmd_enum"
  RollModeSWCmd/2 -> Terminator_48/1
  [BHAL_outputs] -> slr_VHAL_RoomLampMode_flg/1
  slr_VHAL_RoomLampMode_flg/1 -> RoomLampMode/1  "<VHAL_RoomLampMode_flg>"
  True_VHAL_RoomLampMode_flg/1 -> RoomLampMode/2
  [inp_CanValid_bus] -> slr1_49/1
  slr1_49/1 -> RoomLampMode/3  "<VINP_CANMsgValidIVI2_flg>"
  RoomLampMode/1 -> VINP_RoomLampMode_flg/1  "VINP_RoomLampMode_flg"
  RoomLampMode/2 -> Terminator_49/1
  [BHAL_outputs] -> slr_VHAL_SOCADJBUTT_flg/1
  slr_VHAL_SOCADJBUTT_flg/1 -> SOCADJBUTT/1  "<VHAL_SOCADJBUTT_flg>"
  True_VHAL_SOCADJBUTT_flg/1 -> SOCADJBUTT/2
  [inp_CanValid_bus] -> slr1_50/1
  slr1_50/1 -> SOCADJBUTT/3  "<VINP_CANMsgValidIVI2_flg>"
  SOCADJBUTT/1 -> VINP_SOCADJBUTT_flg/1  "VINP_SOCADJBUTT_flg"
  SOCADJBUTT/2 -> Terminator_50/1
  [BHAL_outputs] -> slr_VHAL_SOCLimitSet_pct/1
  slr_VHAL_SOCLimitSet_pct/1 -> SOCLimitSet/1  "<VHAL_SOCLimitSet_pct>"
  True_VHAL_SOCLimitSet_pct/1 -> SOCLimitSet/2
  [inp_CanValid_bus] -> slr1_51/1
  slr1_51/1 -> SOCLimitSet/3  "<VINP_CANMsgValidIVI2_flg>"
  SOCLimitSet/1 -> VINP_SOCLimitSet_pct/1  "VINP_SOCLimitSet_pct"
  SOCLimitSet/2 -> Terminator_51/1
  [BHAL_outputs] -> slr_VHAL_SOCV2LLimit_pct/1
  slr_VHAL_SOCV2LLimit_pct/1 -> SOCV2LLimit/1  "<VHAL_SOCV2LLimit_pct>"
  True_VHAL_SOCV2LLimit_pct/1 -> SOCV2LLimit/2
  [inp_CanValid_bus] -> slr1_52/1
  slr1_52/1 -> SOCV2LLimit/3  "<VINP_CANMsgValidIVI2_flg>"
  SOCV2LLimit/1 -> VINP_SOCV2LLimit_pct/1  "VINP_SOCV2LLimit_pct"
  SOCV2LLimit/2 -> Terminator_52/1
  [BHAL_outputs] -> slr_VHAL_SchedChgStart_flg/1
  slr_VHAL_SchedChgStart_flg/1 -> SchedChgStart/1  "<VHAL_SchedChgStart_flg>"
  True_VHAL_SchedChgStart_flg/1 -> SchedChgStart/2
  [inp_CanValid_bus] -> slr1_53/1
  slr1_53/1 -> SchedChgStart/3  "<VINP_CANMsgValidIVI2_flg>"
  SchedChgStart/1 -> VINP_SchedChgStart_flg/1  "VINP_SchedChgStart_flg"
  SchedChgStart/2 -> Terminator_53/1
  [BHAL_outputs] -> slr_VHAL_SchedChgStop_flg/1
  slr_VHAL_SchedChgStop_flg/1 -> SchedChgStop/1  "<VHAL_SchedChgStop_flg>"
  True_VHAL_SchedChgStop_flg/1 -> SchedChgStop/2
  [inp_CanValid_bus] -> slr1_54/1
  slr1_54/1 -> SchedChgStop/3  "<VINP_CANMsgValidIVI2_flg>"
  SchedChgStop/1 -> VINP_SchedChgStop_flg/1  "VINP_SchedChgStop_flg"
  SchedChgStop/2 -> Terminator_54/1
  [BHAL_outputs] -> slr_VHAL_SchedChgbutt_flg/1
  slr_VHAL_SchedChgbutt_flg/1 -> SchedChgbutt/1  "<VHAL_SchedChgbutt_flg>"
  True_VHAL_SchedChgbutt_flg/1 -> SchedChgbutt/2
  [inp_CanValid_bus] -> slr1_55/1
  slr1_55/1 -> SchedChgbutt/3  "<VINP_CANMsgValidIVI2_flg>"
  SchedChgbutt/1 -> VINP_SchedChgbutt_flg/1  "VINP_SchedChgbutt_flg"
  SchedChgbutt/2 -> Terminator_55/1
  [BHAL_outputs] -> slr_VHAL_SchedChglimit_pct/1
  slr_VHAL_SchedChglimit_pct/1 -> SchedChglimit/1  "<VHAL_SchedChglimit_pct>"
  True_VHAL_SchedChglimit_pct/1 -> SchedChglimit/2
  [inp_CanValid_bus] -> slr1_56/1
  slr1_56/1 -> SchedChglimit/3  "<VINP_CANMsgValidIVI2_flg>"
  SchedChglimit/1 -> VINP_SchedChglimit_pct/1  "VINP_SchedChglimit_pct"
  SchedChglimit/2 -> Terminator_56/1
  [BHAL_outputs] -> slr_VHAL_SchedChgwake_flg/1
  slr_VHAL_SchedChgwake_flg/1 -> SchedChgwake/1  "<VHAL_SchedChgwake_flg>"
  True_VHAL_SchedChgwake_flg/1 -> SchedChgwake/2
  [inp_CanValid_bus] -> slr1_57/1
  slr1_57/1 -> SchedChgwake/3  "<VINP_CANMsgValidIVI2_flg>"
  SchedChgwake/1 -> VINP_SchedChgwake_flg/1  "VINP_SchedChgwake_flg"
  SchedChgwake/2 -> Terminator_57/1
  [BHAL_outputs] -> slr_VHAL_SenstivityPosition_enum/1
  slr_VHAL_SenstivityPosition_enum/1 -> SenstivityPosition/1  "<VHAL_SenstivityPosition_enum>"
  True_VHAL_SenstivityPosition_enum/1 -> SenstivityPosition/2
  [inp_CanValid_bus] -> slr1_58/1
  slr1_58/1 -> SenstivityPosition/3  "<VINP_CANMsgValidIVI2_flg>"
  SenstivityPosition/1 -> VINP_SenstivityPosition_enum/1  "VINP_SenstivityPosition_enum"
  SenstivityPosition/2 -> Terminator_58/1
  [BHAL_outputs] -> slr_VHAL_SetUnlockSingle_flg/1
  slr_VHAL_SetUnlockSingle_flg/1 -> SetUnlockSingle/1  "<VHAL_SetUnlockSingle_flg>"
  True_VHAL_SetUnlockSingle_flg/1 -> SetUnlockSingle/2
  [inp_CanValid_bus] -> slr1_59/1
  slr1_59/1 -> SetUnlockSingle/3  "<VINP_CANMsgValidIVI2_flg>"
  SetUnlockSingle/1 -> VINP_SetUnlockSingle_flg/1  "VINP_SetUnlockSingle_flg"
  SetUnlockSingle/2 -> Terminator_59/1
  [BHAL_outputs] -> slr_VHAL_TCSSWCmd_enum/1
  slr_VHAL_TCSSWCmd_enum/1 -> TCSSWCmd/1  "<VHAL_TCSSWCmd_enum>"
  True_VHAL_TCSSWCmd_enum/1 -> TCSSWCmd/2
  [inp_CanValid_bus] -> slr1_60/1
  slr1_60/1 -> TCSSWCmd/3  "<VINP_CANMsgValidIVI2_flg>"
  TCSSWCmd/1 -> VINP_TCSSWCmd_enum/1  "VINP_TCSSWCmd_enum"
  TCSSWCmd/2 -> Terminator_60/1
  [BHAL_outputs] -> slr_VHAL_TPMSCaliButt_flg/1
  slr_VHAL_TPMSCaliButt_flg/1 -> TPMSCaliButt/1  "<VHAL_TPMSCaliButt_flg>"
  True_VHAL_TPMSCaliButt_flg/1 -> TPMSCaliButt/2
  [inp_CanValid_bus] -> slr1_61/1
  slr1_61/1 -> TPMSCaliButt/3  "<VINP_CANMsgValidIVI2_flg>"
  TPMSCaliButt/1 -> VINP_TPMSCaliButt_flg/1  "VINP_TPMSCaliButt_flg"
  TPMSCaliButt/2 -> Terminator_61/1
  [BHAL_outputs] -> slr_VHAL_TPMSResButt_flg/1
  slr_VHAL_TPMSResButt_flg/1 -> TPMSResButt/1  "<VHAL_TPMSResButt_flg>"
  True_VHAL_TPMSResButt_flg/1 -> TPMSResButt/2
  [inp_CanValid_bus] -> slr1_62/1
  slr1_62/1 -> TPMSResButt/3  "<VINP_CANMsgValidIVI2_flg>"
  TPMSResButt/1 -> VINP_TPMSResButt_flg/1  "VINP_TPMSResButt_flg"
  TPMSResButt/2 -> Terminator_62/1
  [BHAL_outputs] -> slr_VHAL_TurnSwTimeSet_enum/1
  slr_VHAL_TurnSwTimeSet_enum/1 -> TurnSwTimeSet/1  "<VHAL_TurnSwTimeSet_enum>"
  True_VHAL_TurnSwTimeSet_enum/1 -> TurnSwTimeSet/2
  [inp_CanValid_bus] -> slr1_63/1
  slr1_63/1 -> TurnSwTimeSet/3  "<VINP_CANMsgValidIVI2_flg>"
  TurnSwTimeSet/1 -> VINP_TurnSwTimeSet_enum/1  "VINP_TurnSwTimeSet_enum"
  TurnSwTimeSet/2 -> Terminator_63/1
  [BHAL_outputs] -> slr_VHAL_WalkawayLockSW_flg/1
  slr_VHAL_WalkawayLockSW_flg/1 -> WalkawayLockSW/1  "<VHAL_WalkawayLockSW_flg>"
  True_VHAL_WalkawayLockSW_flg/1 -> WalkawayLockSW/2
  [inp_CanValid_bus] -> slr1_64/1
  slr1_64/1 -> WalkawayLockSW/3  "<VINP_CANMsgValidIVI2_flg>"
  WalkawayLockSW/1 -> VINP_WalkawayLockSW_flg/1  "VINP_WalkawayLockSW_flg"
  WalkawayLockSW/2 -> Terminator_64/1
  [BHAL_outputs] -> slr_VHAL_WlcmLightMode_enum/1
  slr_VHAL_WlcmLightMode_enum/1 -> WlcmLightMode/1  "<VHAL_WlcmLightMode_enum>"
  True_VHAL_WlcmLightMode_enum/1 -> WlcmLightMode/2
  [inp_CanValid_bus] -> slr1_65/1
  slr1_65/1 -> WlcmLightMode/3  "<VINP_CANMsgValidIVI2_flg>"
  WlcmLightMode/1 -> VINP_WlcmLightMode_enum/1  "VINP_WlcmLightMode_enum"
  WlcmLightMode/2 -> Terminator_65/1
  [BHAL_outputs] -> slr_VHAL_sigAirIntenZon1Req_enum/1
  slr_VHAL_sigAirIntenZon1Req_enum/1 -> sigAirIntenZon1Req/1  "<VHAL_sigAirIntenZon1Req_enum>"
  True_VHAL_sigAirIntenZon1Req_enum/1 -> sigAirIntenZon1Req/2
  [inp_CanValid_bus] -> slr1_66/1
  slr1_66/1 -> sigAirIntenZon1Req/3  "<VINP_CANMsgValidIVI2_flg>"
  sigAirIntenZon1Req/1 -> VINP_sigAirIntenZon1Req_enum/1  "VINP_sigAirIntenZon1Req_enum"
  sigAirIntenZon1Req/2 -> Terminator_66/1
  [BHAL_outputs] -> slr_VHAL_sigDfrstReq_flg/1
  slr_VHAL_sigDfrstReq_flg/1 -> sigDfrstReq/1  "<VHAL_sigDfrstReq_flg>"
  True_VHAL_sigDfrstReq_flg/1 -> sigDfrstReq/2
  [inp_CanValid_bus] -> slr1_67/1
  slr1_67/1 -> sigDfrstReq/3  "<VINP_CANMsgValidIVI2_flg>"
  sigDfrstReq/1 -> VINP_sigDfrstReq_flg/1  "VINP_sigDfrstReq_flg"
  sigDfrstReq/2 -> Terminator_67/1
  [BHAL_outputs] -> slr_VHAL_sigFaceReq_flg/1
  slr_VHAL_sigFaceReq_flg/1 -> sigFaceReq/1  "<VHAL_sigFaceReq_flg>"
  True_VHAL_sigFaceReq_flg/1 -> sigFaceReq/2
  [inp_CanValid_bus] -> slr1_68/1
  slr1_68/1 -> sigFaceReq/3  "<VINP_CANMsgValidIVI2_flg>"
  sigFaceReq/1 -> VINP_sigFaceReq_flg/1  "VINP_sigFaceReq_flg"
  sigFaceReq/2 -> Terminator_68/1
  [BHAL_outputs] -> slr_VHAL_sigFootReq_flg/1
  slr_VHAL_sigFootReq_flg/1 -> sigFootReq/1  "<VHAL_sigFootReq_flg>"
  True_VHAL_sigFootReq_flg/1 -> sigFootReq/2
  [inp_CanValid_bus] -> slr1_69/1
  slr1_69/1 -> sigFootReq/3  "<VINP_CANMsgValidIVI2_flg>"
  sigFootReq/1 -> VINP_sigFootReq_flg/1  "VINP_sigFootReq_flg"
  sigFootReq/2 -> Terminator_69/1
  [BHAL_outputs] -> slr_VHAL_sigRecircReq_flg/1
  slr_VHAL_sigRecircReq_flg/1 -> sigRecircReq/1  "<VHAL_sigRecircReq_flg>"
  True_VHAL_sigRecircReq_flg/1 -> sigRecircReq/2
  [inp_CanValid_bus] -> slr1_70/1
  slr1_70/1 -> sigRecircReq/3  "<VINP_CANMsgValidIVI2_flg>"
  sigRecircReq/1 -> VINP_sigRecircReq_flg/1  "VINP_sigRecircReq_flg"
  sigRecircReq/2 -> Terminator_70/1
  [BHAL_outputs] -> slr_VHAL_sigSetTempZon1Req_C/1
  slr_VHAL_sigSetTempZon1Req_C/1 -> sigSetTempZon1Req/1  "<VHAL_sigSetTempZon1Req_C>"
  True_VHAL_sigSetTempZon1Req_C/1 -> sigSetTempZon1Req/2
  [inp_CanValid_bus] -> slr1_71/1
  slr1_71/1 -> sigSetTempZon1Req/3  "<VINP_CANMsgValidIVI2_flg>"
  sigSetTempZon1Req/1 -> VINP_sigSetTempZon1Req_C/1  "VINP_sigSetTempZon1Req_C"
  sigSetTempZon1Req/2 -> Terminator_71/1
  [BHAL_outputs] -> slr_VHAL_sigSetTempZon2Req_C/1
  slr_VHAL_sigSetTempZon2Req_C/1 -> sigSetTempZon2Req/1  "<VHAL_sigSetTempZon2Req_C>"
  True_VHAL_sigSetTempZon2Req_C/1 -> sigSetTempZon2Req/2
  [inp_CanValid_bus] -> slr1_72/1
  slr1_72/1 -> sigSetTempZon2Req/3  "<VINP_CANMsgValidIVI2_flg>"
  sigSetTempZon2Req/1 -> VINP_sigSetTempZon2Req_C/1  "VINP_sigSetTempZon2Req_C"
  sigSetTempZon2Req/2 -> Terminator_72/1
